simulink model "x_rx_reorder"  (R2012b)
(part 2 of 28)

      |         error('%d field names specified, but %d binary pts?', numios, length(current_bins));
      |     end
      | end
  pkt_reord_cnt1 : Subsystem  Tag=xps:sw_reg  AncestorBlock=xps_library/software register  mask(swreg){mode=one value, io_dir=To Processor, io_delay=1, sample_period=1, names=reg, bitwidths=32, arith_types=0, bin_pts=0, sim_port=off, show_format=off}
      mask prompts: io_dir "I/O direction"; io_delay "I/O delay"; sample_period "Sample period"; names "Name:"; bitwidths "Bitwidth:"; arith_types "Type (ufix=0, fix=1, bool=2):"; bin_pts "Binary pt:"; sim_port "Provide sim input/output?"; show_format "Print format string?"
      mask init:
      | swreg_init(gcb)
      settings: AttributesFormatString=1output
      mask TypeOptions mode: one value | fields of equal size | fields of arbitrary size
      mask Callback mode: swreg_cb(gcb);
      mask TypeOptions io_dir: To Processor | From Processor
      mask Callback io_dir:
      | mask_enables = get_param(gcb, 'MaskEnables');
      | mask_names = get_param(gcb, 'MaskNames');
      | if strcmp(get_param(gcb, 'io_dir'), 'To Processor'),
      |     mask_enables{ismember(mask_names, 'sample_period')} = 'off';
      | else
      |     mask_enables{ismember(mask_names, 'sample_period')} = 'on';
      | end
      | set_param(gcb, 'MaskEnables', mask_enables);
      mask Callback bitwidths:
      | blk = gcb;
      | mode = get_param(blk, 'mode');
      | current_widths = eval(get_param(blk, 'bitwidths'));
      | if (strcmp(mode, 'one value') || strcmp(mode, 'fields of equal size')) && (length(current_widths) > 1),
      |     error('Only one width may be specified for this mode.');
      | elseif strcmp(mode, 'fields of arbitrary size')
      |     current_names = textscan(strtrim(strrep(strrep(get_param(blk, 'names'), ']', ''), '[', '')), '%s');
      |     current_names = current_names{1};
      |     numios = length(current_names);
      |     if length(current_widths) ~= numios,
      |         error('%d field names specified, but %d widths?', numios, length(current_widths));
      |     end
      | end
      | total_width = 0;
      | for ctr = 1 : length(current_widths),
      |     total_width = total_width + current_widths(ctr);
      | end
      | if total_width > 32,
      |     error('Total width must be 32 or less, set to %d.', total_width);
      | end
      mask Callback arith_types:
      | blk = gcb;
      | mode = get_param(blk, 'mode');
      | current_types = eval(get_param(blk, 'arith_types'));
      | numios = length(current_types);
      | if (strcmp(mode, 'one value') || strcmp(mode, 'fields of equal size')) && (length(current_types) > 1),
      |     error('Only one type may be specified for this mode.');
      | elseif strcmp(mode, 'fields of arbitrary size')
      |     current_names = textscan(strtrim(strrep(strrep(get_param(blk, 'names'), ']', ''), '[', '')), '%s');
      |     current_names = current_names{1};
      |     numios = length(current_names);
      |     if length(current_types) ~= numios,
      |         error('%d field names specified, but %d types?', numios, length(current_types));
      |     end
      | end
      | problem = 0;
      | for ctr = 1 : numios,
      |     t = current_types(ctr);
      |     if (t < 0) || (t > 2),
      |         problem = t;
      |         ctr = numios + 1;
      |     end
      | end
      | if problem ~= 0,
      |     error('Type cannot be %i, must be 0, 1 or 2.', problem);
      | end
      mask Callback bin_pts:
      | blk = gcb;
      | mode = get_param(blk, 'mode');
      | current_bins = eval(get_param(blk, 'bin_pts'));
      | if (strcmp(mode, 'one value') || strcmp(mode, 'fields of equal size')) && (length(current_bins) > 1),
      |     error('Only one binary pt may be specified for this mode.');
      | elseif strcmp(mode, 'fields of arbitrary size')
      |     current_names = textscan(strtrim(strrep(strrep(get_param(blk, 'names'), ']', ''), '[', '')), '%s');
      |     current_names = current_names{1};
      |     numios = length(current_names);
      |     if length(current_bins) ~= numios,
      |         error('%d field names specified, but %d binary pts?', numios, length(current_bins));
      |     end
      | end
  pkt_reord_cnt2 : Subsystem  Tag=xps:sw_reg  AncestorBlock=xps_library/software register  mask(swreg){mode=one value, io_dir=To Processor, io_delay=1, sample_period=1, names=reg, bitwidths=32, arith_types=0, bin_pts=0, sim_port=off, show_format=off}
      mask prompts: io_dir "I/O direction"; io_delay "I/O delay"; sample_period "Sample period"; names "Name:"; bitwidths "Bitwidth:"; arith_types "Type (ufix=0, fix=1, bool=2):"; bin_pts "Binary pt:"; sim_port "Provide sim input/output?"; show_format "Print format string?"
      mask init:
      | swreg_init(gcb)
      settings: AttributesFormatString=1output
      mask TypeOptions mode: one value | fields of equal size | fields of arbitrary size
      mask Callback mode: swreg_cb(gcb);
      mask TypeOptions io_dir: To Processor | From Processor
      mask Callback io_dir:
      | mask_enables = get_param(gcb, 'MaskEnables');
      | mask_names = get_param(gcb, 'MaskNames');
      | if strcmp(get_param(gcb, 'io_dir'), 'To Processor'),
      |     mask_enables{ismember(mask_names, 'sample_period')} = 'off';
      | else
      |     mask_enables{ismember(mask_names, 'sample_period')} = 'on';
      | end
      | set_param(gcb, 'MaskEnables', mask_enables);
      mask Callback bitwidths:
      | blk = gcb;
      | mode = get_param(blk, 'mode');
      | current_widths = eval(get_param(blk, 'bitwidths'));
      | if (strcmp(mode, 'one value') || strcmp(mode, 'fields of equal size')) && (length(current_widths) > 1),
      |     error('Only one width may be specified for this mode.');
      | elseif strcmp(mode, 'fields of arbitrary size')
      |     current_names = textscan(strtrim(strrep(strrep(get_param(blk, 'names'), ']', ''), '[', '')), '%s');
      |     current_names = current_names{1};
      |     numios = length(current_names);
      |     if length(current_widths) ~= numios,
      |         error('%d field names specified, but %d widths?', numios, length(current_widths));
      |     end
      | end
      | total_width = 0;
      | for ctr = 1 : length(current_widths),
      |     total_width = total_width + current_widths(ctr);
      | end
      | if total_width > 32,
      |     error('Total width must be 32 or less, set to %d.', total_width);
      | end
      mask Callback arith_types:
      | blk = gcb;
      | mode = get_param(blk, 'mode');
      | current_types = eval(get_param(blk, 'arith_types'));
      | numios = length(current_types);
      | if (strcmp(mode, 'one value') || strcmp(mode, 'fields of equal size')) && (length(current_types) > 1),
      |     error('Only one type may be specified for this mode.');
      | elseif strcmp(mode, 'fields of arbitrary size')
      |     current_names = textscan(strtrim(strrep(strrep(get_param(blk, 'names'), ']', ''), '[', '')), '%s');
      |     current_names = current_names{1};
      |     numios = length(current_names);
      |     if length(current_types) ~= numios,
      |         error('%d field names specified, but %d types?', numios, length(current_types));
      |     end
      | end
      | problem = 0;
      | for ctr = 1 : numios,
      |     t = current_types(ctr);
      |     if (t < 0) || (t > 2),
      |         problem = t;
      |         ctr = numios + 1;
      |     end
      | end
      | if problem ~= 0,
      |     error('Type cannot be %i, must be 0, 1 or 2.', problem);
      | end
      mask Callback bin_pts:
      | blk = gcb;
      | mode = get_param(blk, 'mode');
      | current_bins = eval(get_param(blk, 'bin_pts'));
      | if (strcmp(mode, 'one value') || strcmp(mode, 'fields of equal size')) && (length(current_bins) > 1),
      |     error('Only one binary pt may be specified for this mode.');
      | elseif strcmp(mode, 'fields of arbitrary size')
      |     current_names = textscan(strtrim(strrep(strrep(get_param(blk, 'names'), ']', ''), '[', '')), '%s');
      |     current_names = current_names{1};
      |     numios = length(current_names);
      |     if length(current_bins) ~= numios,
      |         error('%d field names specified, but %d binary pts?', numios, length(current_bins));
      |     end
      | end
  pkt_reord_cnt3 : Subsystem  Tag=xps:sw_reg  AncestorBlock=xps_library/software register  mask(swreg){mode=one value, io_dir=To Processor, io_delay=1, sample_period=1, names=reg, bitwidths=32, arith_types=0, bin_pts=0, sim_port=off, show_format=off}
      mask prompts: io_dir "I/O direction"; io_delay "I/O delay"; sample_period "Sample period"; names "Name:"; bitwidths "Bitwidth:"; arith_types "Type (ufix=0, fix=1, bool=2):"; bin_pts "Binary pt:"; sim_port "Provide sim input/output?"; show_format "Print format string?"
      mask init:
      | swreg_init(gcb)
      settings: AttributesFormatString=1output
      mask TypeOptions mode: one value | fields of equal size | fields of arbitrary size
      mask Callback mode: swreg_cb(gcb);
      mask TypeOptions io_dir: To Processor | From Processor
      mask Callback io_dir:
      | mask_enables = get_param(gcb, 'MaskEnables');
      | mask_names = get_param(gcb, 'MaskNames');
      | if strcmp(get_param(gcb, 'io_dir'), 'To Processor'),
      |     mask_enables{ismember(mask_names, 'sample_period')} = 'off';
      | else
      |     mask_enables{ismember(mask_names, 'sample_period')} = 'on';
      | end
      | set_param(gcb, 'MaskEnables', mask_enables);
      mask Callback bitwidths:
      | blk = gcb;
      | mode = get_param(blk, 'mode');
      | current_widths = eval(get_param(blk, 'bitwidths'));
      | if (strcmp(mode, 'one value') || strcmp(mode, 'fields of equal size')) && (length(current_widths) > 1),
      |     error('Only one width may be specified for this mode.');
      | elseif strcmp(mode, 'fields of arbitrary size')
      |     current_names = textscan(strtrim(strrep(strrep(get_param(blk, 'names'), ']', ''), '[', '')), '%s');
      |     current_names = current_names{1};
      |     numios = length(current_names);
      |     if length(current_widths) ~= numios,
      |         error('%d field names specified, but %d widths?', numios, length(current_widths));
      |     end
      | end
      | total_width = 0;
      | for ctr = 1 : length(current_widths),
      |     total_width = total_width + current_widths(ctr);
      | end
      | if total_width > 32,
      |     error('Total width must be 32 or less, set to %d.', total_width);
      | end
      mask Callback arith_types:
      | blk = gcb;
      | mode = get_param(blk, 'mode');
      | current_types = eval(get_param(blk, 'arith_types'));
      | numios = length(current_types);
      | if (strcmp(mode, 'one value') || strcmp(mode, 'fields of equal size')) && (length(current_types) > 1),
      |     error('Only one type may be specified for this mode.');
      | elseif strcmp(mode, 'fields of arbitrary size')
      |     current_names = textscan(strtrim(strrep(strrep(get_param(blk, 'names'), ']', ''), '[', '')), '%s');
      |     current_names = current_names{1};
      |     numios = length(current_names);
      |     if length(current_types) ~= numios,
      |         error('%d field names specified, but %d types?', numios, length(current_types));
      |     end
      | end
      | problem = 0;
      | for ctr = 1 : numios,
      |     t = current_types(ctr);
      |     if (t < 0) || (t > 2),
      |         problem = t;
      |         ctr = numios + 1;
      |     end
      | end
      | if problem ~= 0,
      |     error('Type cannot be %i, must be 0, 1 or 2.', problem);
      | end
      mask Callback bin_pts:
      | blk = gcb;
      | mode = get_param(blk, 'mode');
      | current_bins = eval(get_param(blk, 'bin_pts'));
      | if (strcmp(mode, 'one value') || strcmp(mode, 'fields of equal size')) && (length(current_bins) > 1),
      |     error('Only one binary pt may be specified for this mode.');
      | elseif strcmp(mode, 'fields of arbitrary size')
      |     current_names = textscan(strtrim(strrep(strrep(get_param(blk, 'names'), ']', ''), '[', '')), '%s');
      |     current_names = current_names{1};
      |     numios = length(current_names);
      |     if length(current_bins) ~= numios,
      |         error('%d field names specified, but %d binary pts?', numios, length(current_bins));
      |     end
      | end
  pkt_reord_devel0 : Subsystem  mask{ant_bits=2, xeng_bits=5, chan_bits=12, x_int_bits=8, window_bits=4, min_sync_bits=11}
      mask prompts: ant_bits "Maximum Number of Antennas (2^?):"; xeng_bits "Number of Xengines in the system (2^?)"; chan_bits "Number of frequency channels in the system (2^?)"; x_int_bits "X Engine Integration Length (2^?):"; window_bits "Number of Windows to Buffer (2^?):"; min_sync_bits "Minimum sync period (2^n)"
      mask init:
      | sync_bits=max([min_sync_bits,chan_bits+x_int_bits+ant_bits-xeng_bits]);
      | %sync_bits=chan_bits+x_int_bits+ant_bits-xeng_bits;
      | buf_bits=x_int_bits+ant_bits+window_bits-1; %64b in, 32b out.
      | fmtstr = sprintf('Sync period: 2^%d\nPayload Len: %i', sync_bits, 2^(x_int_bits - 2));
      | set_param(gcb, 'AttributesFormatString', fmtstr);
      settings: AttributesFormatString=|
      | Sync period: 2^17
      | Payload Len: 64
  pkt_reord_devel1 : Subsystem  mask{ant_bits=2, xeng_bits=5, chan_bits=12, x_int_bits=8, window_bits=4, min_sync_bits=11}
      mask prompts: ant_bits "Maximum Number of Antennas (2^?):"; xeng_bits "Number of Xengines in the system (2^?)"; chan_bits "Number of frequency channels in the system (2^?)"; x_int_bits "X Engine Integration Length (2^?):"; window_bits "Number of Windows to Buffer (2^?):"; min_sync_bits "Minimum sync period (2^n)"
      mask init:
      | sync_bits=max([min_sync_bits,chan_bits+x_int_bits+ant_bits-xeng_bits]);
      | %sync_bits=chan_bits+x_int_bits+ant_bits-xeng_bits;
      | buf_bits=x_int_bits+ant_bits+window_bits-1; %64b in, 32b out.
      | fmtstr = sprintf('Sync period: 2^%d\nPayload Len: %i',sync_bits,2^(x_int_bits - 2));
      | set_param(gcb, 'AttributesFormatString', fmtstr);
      settings: AttributesFormatString=|
      | Sync period: 2^17
      | Payload Len: 64
  pkt_reord_devel2 : Subsystem  mask{ant_bits=2, xeng_bits=5, chan_bits=12, x_int_bits=8, window_bits=4, min_sync_bits=11}
      mask prompts: ant_bits "Maximum Number of Antennas (2^?):"; xeng_bits "Number of Xengines in the system (2^?)"; chan_bits "Number of frequency channels in the system (2^?)"; x_int_bits "X Engine Integration Length (2^?):"; window_bits "Number of Windows to Buffer (2^?):"; min_sync_bits "Minimum sync period (2^n)"
      mask init: same as x_rx_reorder/pkt_reord_devel1
      settings: AttributesFormatString=|
      | Sync period: 2^17
      | Payload Len: 64
  pkt_reord_devel3 : Subsystem  mask{ant_bits=2, xeng_bits=5, chan_bits=12, x_int_bits=8, window_bits=4, min_sync_bits=11}
      mask prompts: ant_bits "Maximum Number of Antennas (2^?):"; xeng_bits "Number of Xengines in the system (2^?)"; chan_bits "Number of frequency channels in the system (2^?)"; x_int_bits "X Engine Integration Length (2^?):"; window_bits "Number of Windows to Buffer (2^?):"; min_sync_bits "Minimum sync period (2^n)"
      mask init: same as x_rx_reorder/pkt_reord_devel1
      settings: AttributesFormatString=|
      | Sync period: 2^17
      | Payload Len: 64
  pkt_reord_err0 : Subsystem  Tag=xps:sw_reg  AncestorBlock=xps_library/software register  mask(swreg){mode=one value, io_dir=To Processor, io_delay=1, sample_period=1, names=reg, bitwidths=32, arith_types=0, bin_pts=0, sim_port=off, show_format=off}
      mask prompts: io_dir "I/O direction"; io_delay "I/O delay"; sample_period "Sample period"; names "Name:"; bitwidths "Bitwidth:"; arith_types "Type (ufix=0, fix=1, bool=2):"; bin_pts "Binary pt:"; sim_port "Provide sim input/output?"; show_format "Print format string?"
      mask init:
      | swreg_init(gcb)
      settings: AttributesFormatString=1output
      mask TypeOptions mode: one value | fields of equal size | fields of arbitrary size
      mask Callback mode: swreg_cb(gcb);
      mask TypeOptions io_dir: To Processor | From Processor
      mask Callback io_dir:
      | mask_enables = get_param(gcb, 'MaskEnables');
      | mask_names = get_param(gcb, 'MaskNames');
      | if strcmp(get_param(gcb, 'io_dir'), 'To Processor'),
      |     mask_enables{ismember(mask_names, 'sample_period')} = 'off';
      | else
      |     mask_enables{ismember(mask_names, 'sample_period')} = 'on';
      | end
      | set_param(gcb, 'MaskEnables', mask_enables);
      mask Callback bitwidths:
      | blk = gcb;
      | mode = get_param(blk, 'mode');
      | current_widths = eval(get_param(blk, 'bitwidths'));
      | if (strcmp(mode, 'one value') || strcmp(mode, 'fields of equal size')) && (length(current_widths) > 1),
      |     error('Only one width may be specified for this mode.');
      | elseif strcmp(mode, 'fields of arbitrary size')
      |     current_names = textscan(strtrim(strrep(strrep(get_param(blk, 'names'), ']', ''), '[', '')), '%s');
      |     current_names = current_names{1};
      |     numios = length(current_names);
      |     if length(current_widths) ~= numios,
      |         error('%d field names specified, but %d widths?', numios, length(current_widths));
      |     end
      | end
      | total_width = 0;
      | for ctr = 1 : length(current_widths),
      |     total_width = total_width + current_widths(ctr);
      | end
      | if total_width > 32,
      |     error('Total width must be 32 or less, set to %d.', total_width);
      | end
      mask Callback arith_types:
      | blk = gcb;
      | mode = get_param(blk, 'mode');
      | current_types = eval(get_param(blk, 'arith_types'));
      | numios = length(current_types);
      | if (strcmp(mode, 'one value') || strcmp(mode, 'fields of equal size')) && (length(current_types) > 1),
      |     error('Only one type may be specified for this mode.');
      | elseif strcmp(mode, 'fields of arbitrary size')
      |     current_names = textscan(strtrim(strrep(strrep(get_param(blk, 'names'), ']', ''), '[', '')), '%s');
      |     current_names = current_names{1};
      |     numios = length(current_names);
      |     if length(current_types) ~= numios,
      |         error('%d field names specified, but %d types?', numios, length(current_types));
      |     end
      | end
      | problem = 0;
      | for ctr = 1 : numios,
      |     t = current_types(ctr);
      |     if (t < 0) || (t > 2),
      |         problem = t;
      |         ctr = numios + 1;
      |     end
      | end
      | if problem ~= 0,
      |     error('Type cannot be %i, must be 0, 1 or 2.', problem);
      | end
      mask Callback bin_pts:
      | blk = gcb;
      | mode = get_param(blk, 'mode');
      | current_bins = eval(get_param(blk, 'bin_pts'));
      | if (strcmp(mode, 'one value') || strcmp(mode, 'fields of equal size')) && (length(current_bins) > 1),
      |     error('Only one binary pt may be specified for this mode.');
      | elseif strcmp(mode, 'fields of arbitrary size')
      |     current_names = textscan(strtrim(strrep(strrep(get_param(blk, 'names'), ']', ''), '[', '')), '%s');
      |     current_names = current_names{1};
      |     numios = length(current_names);
      |     if length(current_bins) ~= numios,
      |         error('%d field names specified, but %d binary pts?', numios, length(current_bins));
      |     end
      | end
  pkt_reord_err1 : Subsystem  Tag=xps:sw_reg  AncestorBlock=xps_library/software register  mask(swreg){mode=one value, io_dir=To Processor, io_delay=1, sample_period=1, names=reg, bitwidths=32, arith_types=0, bin_pts=0, sim_port=off, show_format=off}
      mask prompts: io_dir "I/O direction"; io_delay "I/O delay"; sample_period "Sample period"; names "Name:"; bitwidths "Bitwidth:"; arith_types "Type (ufix=0, fix=1, bool=2):"; bin_pts "Binary pt:"; sim_port "Provide sim input/output?"; show_format "Print format string?"
      mask init:
      | swreg_init(gcb)
      settings: AttributesFormatString=1output
      mask TypeOptions mode: one value | fields of equal size | fields of arbitrary size
      mask Callback mode: swreg_cb(gcb);
      mask TypeOptions io_dir: To Processor | From Processor
      mask Callback io_dir:
      | mask_enables = get_param(gcb, 'MaskEnables');
      | mask_names = get_param(gcb, 'MaskNames');
      | if strcmp(get_param(gcb, 'io_dir'), 'To Processor'),
      |     mask_enables{ismember(mask_names, 'sample_period')} = 'off';
      | else
      |     mask_enables{ismember(mask_names, 'sample_period')} = 'on';
      | end
      | set_param(gcb, 'MaskEnables', mask_enables);
      mask Callback bitwidths:
      | blk = gcb;
      | mode = get_param(blk, 'mode');
      | current_widths = eval(get_param(blk, 'bitwidths'));
      | if (strcmp(mode, 'one value') || strcmp(mode, 'fields of equal size')) && (length(current_widths) > 1),
      |     error('Only one width may be specified for this mode.');
      | elseif strcmp(mode, 'fields of arbitrary size')
      |     current_names = textscan(strtrim(strrep(strrep(get_param(blk, 'names'), ']', ''), '[', '')), '%s');
      |     current_names = current_names{1};
      |     numios = length(current_names);
      |     if length(current_widths) ~= numios,
      |         error('%d field names specified, but %d widths?', numios, length(current_widths));
      |     end
      | end
      | total_width = 0;
      | for ctr = 1 : length(current_widths),
      |     total_width = total_width + current_widths(ctr);
      | end
      | if total_width > 32,
      |     error('Total width must be 32 or less, set to %d.', total_width);
      | end
      mask Callback arith_types:
      | blk = gcb;
      | mode = get_param(blk, 'mode');
      | current_types = eval(get_param(blk, 'arith_types'));
      | numios = length(current_types);
      | if (strcmp(mode, 'one value') || strcmp(mode, 'fields of equal size')) && (length(current_types) > 1),
      |     error('Only one type may be specified for this mode.');
      | elseif strcmp(mode, 'fields of arbitrary size')
      |     current_names = textscan(strtrim(strrep(strrep(get_param(blk, 'names'), ']', ''), '[', '')), '%s');
      |     current_names = current_names{1};
      |     numios = length(current_names);
      |     if length(current_types) ~= numios,
      |         error('%d field names specified, but %d types?', numios, length(current_types));
      |     end
      | end
      | problem = 0;
      | for ctr = 1 : numios,
      |     t = current_types(ctr);
      |     if (t < 0) || (t > 2),
      |         problem = t;
      |         ctr = numios + 1;
      |     end
      | end
      | if problem ~= 0,
      |     error('Type cannot be %i, must be 0, 1 or 2.', problem);
      | end
      mask Callback bin_pts:
      | blk = gcb;
      | mode = get_param(blk, 'mode');
      | current_bins = eval(get_param(blk, 'bin_pts'));
      | if (strcmp(mode, 'one value') || strcmp(mode, 'fields of equal size')) && (length(current_bins) > 1),
      |     error('Only one binary pt may be specified for this mode.');
      | elseif strcmp(mode, 'fields of arbitrary size')
      |     current_names = textscan(strtrim(strrep(strrep(get_param(blk, 'names'), ']', ''), '[', '')), '%s');
      |     current_names = current_names{1};
      |     numios = length(current_names);
      |     if length(current_bins) ~= numios,
      |         error('%d field names specified, but %d binary pts?', numios, length(current_bins));
      |     end
      | end
  pkt_reord_err2 : Subsystem  Tag=xps:sw_reg  AncestorBlock=xps_library/software register  mask(swreg){mode=one value, io_dir=To Processor, io_delay=1, sample_period=1, names=reg, bitwidths=32, arith_types=0, bin_pts=0, sim_port=off, show_format=off}
      mask prompts: io_dir "I/O direction"; io_delay "I/O delay"; sample_period "Sample period"; names "Name:"; bitwidths "Bitwidth:"; arith_types "Type (ufix=0, fix=1, bool=2):"; bin_pts "Binary pt:"; sim_port "Provide sim input/output?"; show_format "Print format string?"
      mask init:
      | swreg_init(gcb)
      settings: AttributesFormatString=1output
      mask TypeOptions mode: one value | fields of equal size | fields of arbitrary size
      mask Callback mode: swreg_cb(gcb);
      mask TypeOptions io_dir: To Processor | From Processor
      mask Callback io_dir:
      | mask_enables = get_param(gcb, 'MaskEnables');
      | mask_names = get_param(gcb, 'MaskNames');
      | if strcmp(get_param(gcb, 'io_dir'), 'To Processor'),
      |     mask_enables{ismember(mask_names, 'sample_period')} = 'off';
      | else
      |     mask_enables{ismember(mask_names, 'sample_period')} = 'on';
      | end
      | set_param(gcb, 'MaskEnables', mask_enables);
      mask Callback bitwidths:
      | blk = gcb;
      | mode = get_param(blk, 'mode');
      | current_widths = eval(get_param(blk, 'bitwidths'));
      | if (strcmp(mode, 'one value') || strcmp(mode, 'fields of equal size')) && (length(current_widths) > 1),
      |     error('Only one width may be specified for this mode.');
      | elseif strcmp(mode, 'fields of arbitrary size')
      |     current_names = textscan(strtrim(strrep(strrep(get_param(blk, 'names'), ']', ''), '[', '')), '%s');
      |     current_names = current_names{1};
      |     numios = length(current_names);
      |     if length(current_widths) ~= numios,
      |         error('%d field names specified, but %d widths?', numios, length(current_widths));
      |     end
      | end
      | total_width = 0;
      | for ctr = 1 : length(current_widths),
      |     total_width = total_width + current_widths(ctr);
      | end
      | if total_width > 32,
      |     error('Total width must be 32 or less, set to %d.', total_width);
      | end
      mask Callback arith_types:
      | blk = gcb;
      | mode = get_param(blk, 'mode');
      | current_types = eval(get_param(blk, 'arith_types'));
      | numios = length(current_types);
      | if (strcmp(mode, 'one value') || strcmp(mode, 'fields of equal size')) && (length(current_types) > 1),
      |     error('Only one type may be specified for this mode.');
      | elseif strcmp(mode, 'fields of arbitrary size')
      |     current_names = textscan(strtrim(strrep(strrep(get_param(blk, 'names'), ']', ''), '[', '')), '%s');
      |     current_names = current_names{1};
      |     numios = length(current_names);
      |     if length(current_types) ~= numios,
      |         error('%d field names specified, but %d types?', numios, length(current_types));
      |     end
      | end
      | problem = 0;
      | for ctr = 1 : numios,
      |     t = current_types(ctr);
      |     if (t < 0) || (t > 2),
      |         problem = t;
      |         ctr = numios + 1;
      |     end
      | end
      | if problem ~= 0,
      |     error('Type cannot be %i, must be 0, 1 or 2.', problem);
      | end
      mask Callback bin_pts:
      | blk = gcb;
      | mode = get_param(blk, 'mode');
      | current_bins = eval(get_param(blk, 'bin_pts'));
      | if (strcmp(mode, 'one value') || strcmp(mode, 'fields of equal size')) && (length(current_bins) > 1),
      |     error('Only one binary pt may be specified for this mode.');
      | elseif strcmp(mode, 'fields of arbitrary size')
      |     current_names = textscan(strtrim(strrep(strrep(get_param(blk, 'names'), ']', ''), '[', '')), '%s');
      |     current_names = current_names{1};
      |     numios = length(current_names);
      |     if length(current_bins) ~= numios,
      |         error('%d field names specified, but %d binary pts?', numios, length(current_bins));
      |     end
      | end
  pkt_reord_err3 : Subsystem  Tag=xps:sw_reg  AncestorBlock=xps_library/software register  mask(swreg){mode=one value, io_dir=To Processor, io_delay=1, sample_period=1, names=reg, bitwidths=32, arith_types=0, bin_pts=0, sim_port=off, show_format=off}
      mask prompts: io_dir "I/O direction"; io_delay "I/O delay"; sample_period "Sample period"; names "Name:"; bitwidths "Bitwidth:"; arith_types "Type (ufix=0, fix=1, bool=2):"; bin_pts "Binary pt:"; sim_port "Provide sim input/output?"; show_format "Print format string?"
      mask init:
      | swreg_init(gcb)
      settings: AttributesFormatString=1output
      mask TypeOptions mode: one value | fields of equal size | fields of arbitrary size
      mask Callback mode: swreg_cb(gcb);
      mask TypeOptions io_dir: To Processor | From Processor
      mask Callback io_dir:
      | mask_enables = get_param(gcb, 'MaskEnables');
      | mask_names = get_param(gcb, 'MaskNames');
      | if strcmp(get_param(gcb, 'io_dir'), 'To Processor'),
      |     mask_enables{ismember(mask_names, 'sample_period')} = 'off';
      | else
      |     mask_enables{ismember(mask_names, 'sample_period')} = 'on';
      | end
      | set_param(gcb, 'MaskEnables', mask_enables);
      mask Callback bitwidths:
      | blk = gcb;
      | mode = get_param(blk, 'mode');
      | current_widths = eval(get_param(blk, 'bitwidths'));
      | if (strcmp(mode, 'one value') || strcmp(mode, 'fields of equal size')) && (length(current_widths) > 1),
      |     error('Only one width may be specified for this mode.');
      | elseif strcmp(mode, 'fields of arbitrary size')
      |     current_names = textscan(strtrim(strrep(strrep(get_param(blk, 'names'), ']', ''), '[', '')), '%s');
      |     current_names = current_names{1};
      |     numios = length(current_names);
      |     if length(current_widths) ~= numios,
      |         error('%d field names specified, but %d widths?', numios, length(current_widths));
      |     end
      | end
      | total_width = 0;
      | for ctr = 1 : length(current_widths),
      |     total_width = total_width + current_widths(ctr);
      | end
      | if total_width > 32,
      |     error('Total width must be 32 or less, set to %d.', total_width);
      | end
      mask Callback arith_types:
      | blk = gcb;
      | mode = get_param(blk, 'mode');
      | current_types = eval(get_param(blk, 'arith_types'));
      | numios = length(current_types);
      | if (strcmp(mode, 'one value') || strcmp(mode, 'fields of equal size')) && (length(current_types) > 1),
      |     error('Only one type may be specified for this mode.');
      | elseif strcmp(mode, 'fields of arbitrary size')
      |     current_names = textscan(strtrim(strrep(strrep(get_param(blk, 'names'), ']', ''), '[', '')), '%s');
      |     current_names = current_names{1};
      |     numios = length(current_names);
      |     if length(current_types) ~= numios,
      |         error('%d field names specified, but %d types?', numios, length(current_types));
      |     end
      | end
      | problem = 0;
      | for ctr = 1 : numios,
      |     t = current_types(ctr);
      |     if (t < 0) || (t > 2),
      |         problem = t;
      |         ctr = numios + 1;
      |     end
      | end
      | if problem ~= 0,
      |     error('Type cannot be %i, must be 0, 1 or 2.', problem);
      | end
      mask Callback bin_pts:
      | blk = gcb;
      | mode = get_param(blk, 'mode');
      | current_bins = eval(get_param(blk, 'bin_pts'));
      | if (strcmp(mode, 'one value') || strcmp(mode, 'fields of equal size')) && (length(current_bins) > 1),
      |     error('Only one binary pt may be specified for this mode.');
      | elseif strcmp(mode, 'fields of arbitrary size')
      |     current_names = textscan(strtrim(strrep(strrep(get_param(blk, 'names'), ']', ''), '[', '')), '%s');
      |     current_names = current_names{1};
      |     numios = length(current_names);
      |     if length(current_bins) ~= numios,
      |         error('%d field names specified, but %d binary pts?', numios, length(current_bins));
      |     end
      | end
  pre_process0 : Subsystem  mask{share_bits=1, xeng_bits=5, freq_bits=12}
      mask prompts: share_bits "Number of X-engines on this link (2^N)?"; xeng_bits "Number of X-engines in system (2^N)?"; freq_bits "Number of frequency channels in system (2^N)?"
  pre_process1 : Subsystem  mask{share_bits=1, xeng_bits=5, freq_bits=12}
      mask prompts: share_bits "Number of X-engines on this link (2^N)?"; xeng_bits "Number of X-engines in system (2^N)?"; freq_bits "Number of frequency channels in system (2^N)?"
  pre_process2 : Subsystem  mask{share_bits=1, xeng_bits=5, freq_bits=12}
      mask prompts: share_bits "Number of X-engines on this link (2^N)?"; xeng_bits "Number of X-engines in system (2^N)?"; freq_bits "Number of frequency channels in system (2^N)?"
  pre_process3 : Subsystem  mask{share_bits=1, xeng_bits=5, freq_bits=12}
      mask prompts: share_bits "Number of X-engines on this link (2^N)?"; xeng_bits "Number of X-engines in system (2^N)?"; freq_bits "Number of frequency channels in system (2^N)?"
  rx_cnt0 : Subsystem  Tag=xps:sw_reg  AncestorBlock=xps_library/software register  mask(swreg){mode=one value, io_dir=To Processor, io_delay=1, sample_period=1, names=reg, bitwidths=32, arith_types=0, bin_pts=0, sim_port=off, show_format=off}
      mask prompts: io_dir "I/O direction"; io_delay "I/O delay"; sample_period "Sample period"; names "Name:"; bitwidths "Bitwidth:"; arith_types "Type (ufix=0, fix=1, bool=2):"; bin_pts "Binary pt:"; sim_port "Provide sim input/output?"; show_format "Print format string?"
      mask init:
      | swreg_init(gcb)
      settings: AttributesFormatString=1output
      mask TypeOptions mode: one value | fields of equal size | fields of arbitrary size
      mask Callback mode: swreg_cb(gcb);
      mask TypeOptions io_dir: To Processor | From Processor
      mask Callback io_dir:
      | mask_enables = get_param(gcb, 'MaskEnables');
      | mask_names = get_param(gcb, 'MaskNames');
      | if strcmp(get_param(gcb, 'io_dir'), 'To Processor'),
      |     mask_enables{ismember(mask_names, 'sample_period')} = 'off';
      | else
      |     mask_enables{ismember(mask_names, 'sample_period')} = 'on';
      | end
      | set_param(gcb, 'MaskEnables', mask_enables);
      mask Callback bitwidths:
      | blk = gcb;
      | mode = get_param(blk, 'mode');
      | current_widths = eval(get_param(blk, 'bitwidths'));
      | if (strcmp(mode, 'one value') || strcmp(mode, 'fields of equal size')) && (length(current_widths) > 1),
      |     error('Only one width may be specified for this mode.');
      | elseif strcmp(mode, 'fields of arbitrary size')
      |     current_names = textscan(strtrim(strrep(strrep(get_param(blk, 'names'), ']', ''), '[', '')), '%s');
      |     current_names = current_names{1};
      |     numios = length(current_names);
      |     if length(current_widths) ~= numios,
      |         error('%d field names specified, but %d widths?', numios, length(current_widths));
      |     end
      | end
      | total_width = 0;
      | for ctr = 1 : length(current_widths),
      |     total_width = total_width + current_widths(ctr);
      | end
      | if total_width > 32,
      |     error('Total width must be 32 or less, set to %d.', total_width);
      | end
      mask Callback arith_types:
      | blk = gcb;
      | mode = get_param(blk, 'mode');
      | current_types = eval(get_param(blk, 'arith_types'));
      | numios = length(current_types);
      | if (strcmp(mode, 'one value') || strcmp(mode, 'fields of equal size')) && (length(current_types) > 1),
      |     error('Only one type may be specified for this mode.');
      | elseif strcmp(mode, 'fields of arbitrary size')
      |     current_names = textscan(strtrim(strrep(strrep(get_param(blk, 'names'), ']', ''), '[', '')), '%s');
      |     current_names = current_names{1};
      |     numios = length(current_names);
      |     if length(current_types) ~= numios,
      |         error('%d field names specified, but %d types?', numios, length(current_types));
      |     end
      | end
      | problem = 0;
      | for ctr = 1 : numios,
      |     t = current_types(ctr);
      |     if (t < 0) || (t > 2),
      |         problem = t;
      |         ctr = numios + 1;
      |     end
      | end
      | if problem ~= 0,
      |     error('Type cannot be %i, must be 0, 1 or 2.', problem);
      | end
      mask Callback bin_pts:
      | blk = gcb;
      | mode = get_param(blk, 'mode');
      | current_bins = eval(get_param(blk, 'bin_pts'));
      | if (strcmp(mode, 'one value') || strcmp(mode, 'fields of equal size')) && (length(current_bins) > 1),
      |     error('Only one binary pt may be specified for this mode.');
      | elseif strcmp(mode, 'fields of arbitrary size')
      |     current_names = textscan(strtrim(strrep(strrep(get_param(blk, 'names'), ']', ''), '[', '')), '%s');
      |     current_names = current_names{1};
      |     numios = length(current_names);
      |     if length(current_bins) ~= numios,
      |         error('%d field names specified, but %d binary pts?', numios, length(current_bins));
      |     end
      | end
  rx_cnt1 : Subsystem  Tag=xps:sw_reg  AncestorBlock=xps_library/software register  mask(swreg){mode=one value, io_dir=To Processor, io_delay=1, sample_period=1, names=reg, bitwidths=32, arith_types=0, bin_pts=0, sim_port=off, show_format=off}
      mask prompts: io_dir "I/O direction"; io_delay "I/O delay"; sample_period "Sample period"; names "Name:"; bitwidths "Bitwidth:"; arith_types "Type (ufix=0, fix=1, bool=2):"; bin_pts "Binary pt:"; sim_port "Provide sim input/output?"; show_format "Print format string?"
      mask init:
      | swreg_init(gcb)
      settings: AttributesFormatString=1output
      mask TypeOptions mode: one value | fields of equal size | fields of arbitrary size
      mask Callback mode: swreg_cb(gcb);
      mask TypeOptions io_dir: To Processor | From Processor
      mask Callback io_dir:
      | mask_enables = get_param(gcb, 'MaskEnables');
      | mask_names = get_param(gcb, 'MaskNames');
      | if strcmp(get_param(gcb, 'io_dir'), 'To Processor'),
      |     mask_enables{ismember(mask_names, 'sample_period')} = 'off';
      | else
      |     mask_enables{ismember(mask_names, 'sample_period')} = 'on';
      | end
      | set_param(gcb, 'MaskEnables', mask_enables);
      mask Callback bitwidths:
      | blk = gcb;
      | mode = get_param(blk, 'mode');
      | current_widths = eval(get_param(blk, 'bitwidths'));
      | if (strcmp(mode, 'one value') || strcmp(mode, 'fields of equal size')) && (length(current_widths) > 1),
      |     error('Only one width may be specified for this mode.');
      | elseif strcmp(mode, 'fields of arbitrary size')
      |     current_names = textscan(strtrim(strrep(strrep(get_param(blk, 'names'), ']', ''), '[', '')), '%s');
      |     current_names = current_names{1};
      |     numios = length(current_names);
      |     if length(current_widths) ~= numios,
      |         error('%d field names specified, but %d widths?', numios, length(current_widths));
      |     end
      | end
      | total_width = 0;
      | for ctr = 1 : length(current_widths),
      |     total_width = total_width + current_widths(ctr);
      | end
      | if total_width > 32,
      |     error('Total width must be 32 or less, set to %d.', total_width);
      | end
      mask Callback arith_types:
      | blk = gcb;
      | mode = get_param(blk, 'mode');
      | current_types = eval(get_param(blk, 'arith_types'));
      | numios = length(current_types);
      | if (strcmp(mode, 'one value') || strcmp(mode, 'fields of equal size')) && (length(current_types) > 1),
      |     error('Only one type may be specified for this mode.');
      | elseif strcmp(mode, 'fields of arbitrary size')
      |     current_names = textscan(strtrim(strrep(strrep(get_param(blk, 'names'), ']', ''), '[', '')), '%s');
      |     current_names = current_names{1};
      |     numios = length(current_names);
      |     if length(current_types) ~= numios,
      |         error('%d field names specified, but %d types?', numios, length(current_types));
      |     end
      | end
      | problem = 0;
      | for ctr = 1 : numios,
      |     t = current_types(ctr);
      |     if (t < 0) || (t > 2),
      |         problem = t;
      |         ctr = numios + 1;
      |     end
      | end
      | if problem ~= 0,
      |     error('Type cannot be %i, must be 0, 1 or 2.', problem);
      | end
      mask Callback bin_pts:
      | blk = gcb;
      | mode = get_param(blk, 'mode');
      | current_bins = eval(get_param(blk, 'bin_pts'));
      | if (strcmp(mode, 'one value') || strcmp(mode, 'fields of equal size')) && (length(current_bins) > 1),
      |     error('Only one binary pt may be specified for this mode.');
      | elseif strcmp(mode, 'fields of arbitrary size')
      |     current_names = textscan(strtrim(strrep(strrep(get_param(blk, 'names'), ']', ''), '[', '')), '%s');
      |     current_names = current_names{1};
      |     numios = length(current_names);
      |     if length(current_bins) ~= numios,
      |         error('%d field names specified, but %d binary pts?', numios, length(current_bins));
      |     end
      | end
  rx_err_cnt0 : Subsystem  Tag=xps:sw_reg  AncestorBlock=xps_library/software register  mask(swreg){mode=one value, io_dir=To Processor, io_delay=1, sample_period=1, names=reg, bitwidths=32, arith_types=0, bin_pts=0, sim_port=off, show_format=off}
      mask prompts: io_dir "I/O direction"; io_delay "I/O delay"; sample_period "Sample period"; names "Name:"; bitwidths "Bitwidth:"; arith_types "Type (ufix=0, fix=1, bool=2):"; bin_pts "Binary pt:"; sim_port "Provide sim input/output?"; show_format "Print format string?"
      mask init:
      | swreg_init(gcb)
      settings: AttributesFormatString=1output
      mask TypeOptions mode: one value | fields of equal size | fields of arbitrary size
      mask Callback mode: swreg_cb(gcb);
      mask TypeOptions io_dir: To Processor | From Processor
      mask Callback io_dir:
      | mask_enables = get_param(gcb, 'MaskEnables');
      | mask_names = get_param(gcb, 'MaskNames');
      | if strcmp(get_param(gcb, 'io_dir'), 'To Processor'),
      |     mask_enables{ismember(mask_names, 'sample_period')} = 'off';
      | else
      |     mask_enables{ismember(mask_names, 'sample_period')} = 'on';
      | end
      | set_param(gcb, 'MaskEnables', mask_enables);
      mask Callback bitwidths:
      | blk = gcb;
      | mode = get_param(blk, 'mode');
      | current_widths = eval(get_param(blk, 'bitwidths'));
      | if (strcmp(mode, 'one value') || strcmp(mode, 'fields of equal size')) && (length(current_widths) > 1),
      |     error('Only one width may be specified for this mode.');
      | elseif strcmp(mode, 'fields of arbitrary size')
      |     current_names = textscan(strtrim(strrep(strrep(get_param(blk, 'names'), ']', ''), '[', '')), '%s');
      |     current_names = current_names{1};
      |     numios = length(current_names);
      |     if length(current_widths) ~= numios,
      |         error('%d field names specified, but %d widths?', numios, length(current_widths));
      |     end
      | end
      | total_width = 0;
      | for ctr = 1 : length(current_widths),
      |     total_width = total_width + current_widths(ctr);
      | end
      | if total_width > 32,
      |     error('Total width must be 32 or less, set to %d.', total_width);
      | end
      mask Callback arith_types:
      | blk = gcb;
      | mode = get_param(blk, 'mode');
      | current_types = eval(get_param(blk, 'arith_types'));
      | numios = length(current_types);
      | if (strcmp(mode, 'one value') || strcmp(mode, 'fields of equal size')) && (length(current_types) > 1),
      |     error('Only one type may be specified for this mode.');
      | elseif strcmp(mode, 'fields of arbitrary size')
      |     current_names = textscan(strtrim(strrep(strrep(get_param(blk, 'names'), ']', ''), '[', '')), '%s');
      |     current_names = current_names{1};
      |     numios = length(current_names);
      |     if length(current_types) ~= numios,
      |         error('%d field names specified, but %d types?', numios, length(current_types));
      |     end
      | end
      | problem = 0;
      | for ctr = 1 : numios,
      |     t = current_types(ctr);
      |     if (t < 0) || (t > 2),
      |         problem = t;
      |         ctr = numios + 1;
      |     end
      | end
      | if problem ~= 0,
      |     error('Type cannot be %i, must be 0, 1 or 2.', problem);
      | end
      mask Callback bin_pts:
      | blk = gcb;
      | mode = get_param(blk, 'mode');
      | current_bins = eval(get_param(blk, 'bin_pts'));
      | if (strcmp(mode, 'one value') || strcmp(mode, 'fields of equal size')) && (length(current_bins) > 1),
      |     error('Only one binary pt may be specified for this mode.');
      | elseif strcmp(mode, 'fields of arbitrary size')
      |     current_names = textscan(strtrim(strrep(strrep(get_param(blk, 'names'), ']', ''), '[', '')), '%s');
      |     current_names = current_names{1};
      |     numios = length(current_names);
      |     if length(current_bins) ~= numios,
      |         error('%d field names specified, but %d binary pts?', numios, length(current_bins));
      |     end
      | end
  rx_err_cnt1 : Subsystem  Tag=xps:sw_reg  AncestorBlock=xps_library/software register  mask(swreg){mode=one value, io_dir=To Processor, io_delay=1, sample_period=1, names=reg, bitwidths=32, arith_types=0, bin_pts=0, sim_port=off, show_format=off}
      mask prompts: io_dir "I/O direction"; io_delay "I/O delay"; sample_period "Sample period"; names "Name:"; bitwidths "Bitwidth:"; arith_types "Type (ufix=0, fix=1, bool=2):"; bin_pts "Binary pt:"; sim_port "Provide sim input/output?"; show_format "Print format string?"
      mask init:
      | swreg_init(gcb)
      settings: AttributesFormatString=1output
      mask TypeOptions mode: one value | fields of equal size | fields of arbitrary size
      mask Callback mode: swreg_cb(gcb);
      mask TypeOptions io_dir: To Processor | From Processor
      mask Callback io_dir:
      | mask_enables = get_param(gcb, 'MaskEnables');
      | mask_names = get_param(gcb, 'MaskNames');
      | if strcmp(get_param(gcb, 'io_dir'), 'To Processor'),
      |     mask_enables{ismember(mask_names, 'sample_period')} = 'off';
      | else
      |     mask_enables{ismember(mask_names, 'sample_period')} = 'on';
      | end
      | set_param(gcb, 'MaskEnables', mask_enables);
      mask Callback bitwidths:
      | blk = gcb;
      | mode = get_param(blk, 'mode');
      | current_widths = eval(get_param(blk, 'bitwidths'));
      | if (strcmp(mode, 'one value') || strcmp(mode, 'fields of equal size')) && (length(current_widths) > 1),
      |     error('Only one width may be specified for this mode.');
      | elseif strcmp(mode, 'fields of arbitrary size')
      |     current_names = textscan(strtrim(strrep(strrep(get_param(blk, 'names'), ']', ''), '[', '')), '%s');
      |     current_names = current_names{1};
      |     numios = length(current_names);
      |     if length(current_widths) ~= numios,
      |         error('%d field names specified, but %d widths?', numios, length(current_widths));
      |     end
      | end
      | total_width = 0;
      | for ctr = 1 : length(current_widths),
      |     total_width = total_width + current_widths(ctr);
      | end
      | if total_width > 32,
      |     error('Total width must be 32 or less, set to %d.', total_width);
      | end
      mask Callback arith_types:
      | blk = gcb;
      | mode = get_param(blk, 'mode');
      | current_types = eval(get_param(blk, 'arith_types'));
      | numios = length(current_types);
      | if (strcmp(mode, 'one value') || strcmp(mode, 'fields of equal size')) && (length(current_types) > 1),
      |     error('Only one type may be specified for this mode.');
      | elseif strcmp(mode, 'fields of arbitrary size')
      |     current_names = textscan(strtrim(strrep(strrep(get_param(blk, 'names'), ']', ''), '[', '')), '%s');
      |     current_names = current_names{1};
      |     numios = length(current_names);
      |     if length(current_types) ~= numios,
      |         error('%d field names specified, but %d types?', numios, length(current_types));
      |     end
      | end
      | problem = 0;
      | for ctr = 1 : numios,
      |     t = current_types(ctr);
      |     if (t < 0) || (t > 2),
      |         problem = t;
      |         ctr = numios + 1;
      |     end
      | end
      | if problem ~= 0,
      |     error('Type cannot be %i, must be 0, 1 or 2.', problem);
      | end
      mask Callback bin_pts:
      | blk = gcb;
      | mode = get_param(blk, 'mode');
      | current_bins = eval(get_param(blk, 'bin_pts'));
      | if (strcmp(mode, 'one value') || strcmp(mode, 'fields of equal size')) && (length(current_bins) > 1),
      |     error('Only one binary pt may be specified for this mode.');
      | elseif strcmp(mode, 'fields of arbitrary size')
      |     current_names = textscan(strtrim(strrep(strrep(get_param(blk, 'names'), ']', ''), '[', '')), '%s');
      |     current_names = current_names{1};
      |     numios = length(current_names);
      |     if length(current_bins) ~= numios,
      |         error('%d field names specified, but %d binary pts?', numios, length(current_bins));
      |     end
      | end
  snap_reord0 : Subsystem  Tag=casper:bitsnap  AncestorBlock=casper_library_scopes/bitfield snapshot  mask(bitsnap){io_names=[sync, data, valid, time, freq, xeng_err, feng_err, adc_over, nd_on], io_widths=[1,32,1,48,42,1,1,1,1], io_bps=[0,0,0,0,0,0,0,0,0], io_types=[2,0,2,0,0,2,2,2,2], snap_storage=bram, snap_dram_dimm=2, snap_dram_clock=250, snap_nsamples=10, snap_data_width=128, snap_offset=on, snap_circap=on, snap_value=off, snap_use_dsp48=on, snap_delay=0, extra_names=[c d], extra_widths=[30 2], extra_bps=[0 0], extra_types=[0 0]}
      mask prompts: io_names "Names [msb...lsb]"; io_widths "Widths [msb...lsb]"; io_bps "Binary pts [msb...lsb]"; io_types "Data types [msb...lsb], ufix=0, fix=1, bool=2"; snap_storage "Storage medium"; snap_dram_dimm "DRAM dimm"; snap_dram_clock "DRAM clock rate"; snap_nsamples "Number of Samples (2^?)"; snap_data_width "Data width"; snap_offset "Start delay support"; snap_circap "Circular capture support"; snap_value "Extra value capture support"; snap_use_dsp48 "Use DSP48s to implement counters"; snap_delay "Pre-snapshot delay"; extra_names "Names [msb...lsb]"; extra_widths "Widths [msb...lsb]"; extra_bps "Binary pts [msb...lsb]"; extra_types "Data types [msb...lsb], ufix=0, fix=1, bool=2"
      mask help:
      | A wrapped snapshot block. Allows specification of inputs to a snapblock word so the toolflow can automatically set up the scope.
      | See documentation for snapshot for explanation of parameters.
      mask init:
      | bitsnap_init(gcb);
      mask TypeOptions snap_storage: bram | dram
      mask Callback snap_storage: bitsnap_callback();
      mask TypeOptions snap_dram_dimm: 1 | 2 | 3 | 4
      mask TypeOptions snap_dram_clock: 200 | 250 | 266 | 300 | 333
      mask TypeOptions snap_data_width: 8 | 16 | 32 | 64 | 128
      mask Callback snap_value: bitsnap_callback();
  snap_unpack0 : Subsystem  Tag=casper:bitsnap  AncestorBlock=casper_library_scopes/bitfield snapshot  mask(bitsnap){io_names=[data valid eof time feng_id freq adc_over spead_err dest_err fft_err feng_rx_err nd_en chksum_err feng_qdr_err], io_widths=[64,1,1,31,7,16,1,1,1,1,1,1,1,1], io_bps=[0,0,0,0,0,0,0,0,0,0,0,0,0,0], io_types=[0,2,2,0,0,0,2,2,2,2,2,2,2,2], snap_storage=bram, snap_dram_dimm=2, snap_dram_clock=250, snap_nsamples=12, snap_data_width=128, snap_offset=on, snap_circap=on, snap_value=off, snap_use_dsp48=on, snap_delay=0, extra_names=[c d], extra_widths=[30 2], extra_bps=[0 0], extra_types=[0 0]}
      mask prompts: io_names "Names [msb...lsb]"; io_widths "Widths [msb...lsb]"; io_bps "Binary pts [msb...lsb]"; io_types "Data types [msb...lsb], ufix=0, fix=1, bool=2"; snap_storage "Storage medium"; snap_dram_dimm "DRAM dimm"; snap_dram_clock "DRAM clock rate"; snap_nsamples "Number of Samples (2^?)"; snap_data_width "Data width"; snap_offset "Start delay support"; snap_circap "Circular capture support"; snap_value "Extra value capture support"; snap_use_dsp48 "Use DSP48s to implement counters"; snap_delay "Pre-snapshot delay"; extra_names "Names [msb...lsb]"; extra_widths "Widths [msb...lsb]"; extra_bps "Binary pts [msb...lsb]"; extra_types "Data types [msb...lsb], ufix=0, fix=1, bool=2"
      mask help:
      | A wrapped snapshot block. Allows specification of inputs to a snapblock word so the toolflow can automatically set up the scope.
      | See documentation for snapshot for explanation of parameters.
      mask init:
      | bitsnap_init(gcb);
      mask TypeOptions snap_storage: bram | dram
      mask Callback snap_storage: bitsnap_callback();
      mask TypeOptions snap_dram_dimm: 1 | 2 | 3 | 4
      mask TypeOptions snap_dram_clock: 200 | 250 | 266 | 300 | 333
      mask TypeOptions snap_data_width: 8 | 16 | 32 | 64 | 128
      mask Callback snap_value: bitsnap_callback();
  snap_unpack1 : Subsystem  Tag=casper:bitsnap  AncestorBlock=casper_library_scopes/bitfield snapshot  mask(bitsnap){io_names=[data valid eof time feng_id freq adc_over spead_err dest_err fft_err feng_rx_err nd_en chksum_err feng_qdr_err], io_widths=[64,1,1,31,7,16,1,1,1,1,1,1,1,1], io_bps=[0,0,0,0,0,0,0,0,0,0,0,0,0,0], io_types=[0,2,2,0,0,0,2,2,2,2,2,2,2,2], snap_storage=bram, snap_dram_dimm=2, snap_dram_clock=250, snap_nsamples=12, snap_data_width=128, snap_offset=on, snap_circap=on, snap_value=off, snap_use_dsp48=on, snap_delay=0, extra_names=[c d], extra_widths=[30 2], extra_bps=[0 0], extra_types=[0 0]}
      mask prompts: io_names "Names [msb...lsb]"; io_widths "Widths [msb...lsb]"; io_bps "Binary pts [msb...lsb]"; io_types "Data types [msb...lsb], ufix=0, fix=1, bool=2"; snap_storage "Storage medium"; snap_dram_dimm "DRAM dimm"; snap_dram_clock "DRAM clock rate"; snap_nsamples "Number of Samples (2^?)"; snap_data_width "Data width"; snap_offset "Start delay support"; snap_circap "Circular capture support"; snap_value "Extra value capture support"; snap_use_dsp48 "Use DSP48s to implement counters"; snap_delay "Pre-snapshot delay"; extra_names "Names [msb...lsb]"; extra_widths "Widths [msb...lsb]"; extra_bps "Binary pts [msb...lsb]"; extra_types "Data types [msb...lsb], ufix=0, fix=1, bool=2"
      mask help:
      | A wrapped snapshot block. Allows specification of inputs to a snapblock word so the toolflow can automatically set up the scope.
      | See documentation for snapshot for explanation of parameters.
      mask init:
      | bitsnap_init(gcb);
      mask TypeOptions snap_storage: bram | dram
      mask Callback snap_storage: bitsnap_callback();
      mask TypeOptions snap_dram_dimm: 1 | 2 | 3 | 4
      mask TypeOptions snap_dram_clock: 200 | 250 | 266 | 300 | 333
      mask TypeOptions snap_data_width: 8 | 16 | 32 | 64 | 128
      mask Callback snap_value: bitsnap_callback();
  snap_unpack2 : Subsystem  Tag=casper:bitsnap  AncestorBlock=casper_library_scopes/bitfield snapshot  mask(bitsnap){io_names=[data valid eof time feng_id freq adc_over spead_err dest_err fft_err feng_rx_err nd_en chksum_err feng_qdr_err], io_widths=[64,1,1,31,7,16,1,1,1,1,1,1,1,1], io_bps=[0,0,0,0,0,0,0,0,0,0,0,0,0,0], io_types=[0,2,2,0,0,0,2,2,2,2,2,2,2,2], snap_storage=bram, snap_dram_dimm=2, snap_dram_clock=250, snap_nsamples=12, snap_data_width=128, snap_offset=on, snap_circap=on, snap_value=off, snap_use_dsp48=on, snap_delay=0, extra_names=[c d], extra_widths=[30 2], extra_bps=[0 0], extra_types=[0 0]}
      mask prompts: io_names "Names [msb...lsb]"; io_widths "Widths [msb...lsb]"; io_bps "Binary pts [msb...lsb]"; io_types "Data types [msb...lsb], ufix=0, fix=1, bool=2"; snap_storage "Storage medium"; snap_dram_dimm "DRAM dimm"; snap_dram_clock "DRAM clock rate"; snap_nsamples "Number of Samples (2^?)"; snap_data_width "Data width"; snap_offset "Start delay support"; snap_circap "Circular capture support"; snap_value "Extra value capture support"; snap_use_dsp48 "Use DSP48s to implement counters"; snap_delay "Pre-snapshot delay"; extra_names "Names [msb...lsb]"; extra_widths "Widths [msb...lsb]"; extra_bps "Binary pts [msb...lsb]"; extra_types "Data types [msb...lsb], ufix=0, fix=1, bool=2"
      mask help:
      | A wrapped snapshot block. Allows specification of inputs to a snapblock word so the toolflow can automatically set up the scope.
      | See documentation for snapshot for explanation of parameters.
      mask init:
      | bitsnap_init(gcb);
      mask TypeOptions snap_storage: bram | dram
      mask Callback snap_storage: bitsnap_callback();
      mask TypeOptions snap_dram_dimm: 1 | 2 | 3 | 4
      mask TypeOptions snap_dram_clock: 200 | 250 | 266 | 300 | 333
      mask TypeOptions snap_data_width: 8 | 16 | 32 | 64 | 128
      mask Callback snap_value: bitsnap_callback();
  snap_unpack3 : Subsystem  Tag=casper:bitsnap  AncestorBlock=casper_library_scopes/bitfield snapshot  mask(bitsnap){io_names=[data valid eof time feng_id freq adc_over spead_err dest_err fft_err feng_rx_err nd_en chksum_err feng_qdr_err], io_widths=[64,1,1,31,7,16,1,1,1,1,1,1,1,1], io_bps=[0,0,0,0,0,0,0,0,0,0,0,0,0,0], io_types=[0,2,2,0,0,0,2,2,2,2,2,2,2,2], snap_storage=bram, snap_dram_dimm=2, snap_dram_clock=250, snap_nsamples=12, snap_data_width=128, snap_offset=on, snap_circap=on, snap_value=off, snap_use_dsp48=on, snap_delay=0, extra_names=[c d], extra_widths=[30 2], extra_bps=[0 0], extra_types=[0 0]}
      mask prompts: io_names "Names [msb...lsb]"; io_widths "Widths [msb...lsb]"; io_bps "Binary pts [msb...lsb]"; io_types "Data types [msb...lsb], ufix=0, fix=1, bool=2"; snap_storage "Storage medium"; snap_dram_dimm "DRAM dimm"; snap_dram_clock "DRAM clock rate"; snap_nsamples "Number of Samples (2^?)"; snap_data_width "Data width"; snap_offset "Start delay support"; snap_circap "Circular capture support"; snap_value "Extra value capture support"; snap_use_dsp48 "Use DSP48s to implement counters"; snap_delay "Pre-snapshot delay"; extra_names "Names [msb...lsb]"; extra_widths "Widths [msb...lsb]"; extra_bps "Binary pts [msb...lsb]"; extra_types "Data types [msb...lsb], ufix=0, fix=1, bool=2"
      mask help:
      | A wrapped snapshot block. Allows specification of inputs to a snapblock word so the toolflow can automatically set up the scope.
      | See documentation for snapshot for explanation of parameters.
      mask init:
      | bitsnap_init(gcb);
      mask TypeOptions snap_storage: bram | dram
      mask Callback snap_storage: bitsnap_callback();
      mask TypeOptions snap_dram_dimm: 1 | 2 | 3 | 4
      mask TypeOptions snap_dram_clock: 200 | 250 | 266 | 300 | 333
      mask TypeOptions snap_data_width: 8 | 16 | 32 | 64 | 128
      mask Callback snap_value: bitsnap_callback();
  spead_unpack0 : Subsystem  Tag=casper:spead_unpack  AncestorBlock=casper_library_communications/spead_unpack  mask(spead_unpack_mask){payload_length=128, header_ids=[hex2dec('1600'),hex2dec('4101'),hex2dec('4102'), hex2dec('4103')], spead_msw=64, spead_lsw=48, spead_version=4, combine_errors=on}
      mask prompts: payload_length "Payload length in 64-bit words"; header_ids "SPEAD header IDs (decimal)"; spead_msw "SPEAD Flavour (MSw)"; spead_lsw "SPEAD Flavour (LSw)"; spead_version "SPEAD version"; combine_errors "Combine error flags"
      mask help: This block receives a 64-bit-word stream that contains a SPEAD stream. It checks the SPEAD headers are being correctly received. It presents the user with all headers on the first valid cycle of data along with a flag to indicate a header or packet-length error.
      mask init:
      | spead_unpack_init(gcb)
  spead_unpack1 : Subsystem  Tag=casper:spead_unpack  AncestorBlock=casper_library_communications/spead_unpack  mask(spead_unpack_mask){payload_length=128, header_ids=[hex2dec('1600'),hex2dec('4101'),hex2dec('4102'), hex2dec('4103')], spead_msw=64, spead_lsw=48, spead_version=4, combine_errors=on}
      mask prompts: payload_length "Payload length in 64-bit words"; header_ids "SPEAD header IDs (decimal)"; spead_msw "SPEAD Flavour (MSw)"; spead_lsw "SPEAD Flavour (LSw)"; spead_version "SPEAD version"; combine_errors "Combine error flags"
      mask help: This block receives a 64-bit-word stream that contains a SPEAD stream. It checks the SPEAD headers are being correctly received. It presents the user with all headers on the first valid cycle of data along with a flag to indicate a header or packet-length error.
      mask init:
      | spead_unpack_init(gcb)
  tvg_select : Subsystem  Tag=xps:sw_reg  AncestorBlock=xps_library/software register  mask(swreg){mode=fields of arbitrary size, io_dir=From Processor, io_delay=1, sample_period=1, names=[xaui descramble xeng vacc], bitwidths=[1 2 2 6], arith_types=[0 0 0 0], bin_pts=[0 0 0 0], sim_port=off, show_format=off}
      mask prompts: io_dir "I/O direction"; io_delay "I/O delay"; sample_period "Sample period"; names "Names [msb ... lsb]:"; bitwidths "Bitwidths [msb ... lsb]:"; arith_types "Types (ufix=0, fix=1, bool=2) [msb ... lsb]:"; bin_pts "Binary pts [msb ... lsb]:"; sim_port "Provide sim input/output?"; show_format "Print format string?"
      mask init:
      | swreg_init(gcb)
      settings: AttributesFormatString=4 inputs
      mask TypeOptions mode: one value | fields of equal size | fields of arbitrary size
      mask Callback mode: swreg_cb(gcb);
      mask TypeOptions io_dir: To Processor | From Processor
      mask Callback io_dir:
      | mask_enables = get_param(gcb, 'MaskEnables');
      | mask_names = get_param(gcb, 'MaskNames');
      | if strcmp(get_param(gcb, 'io_dir'), 'To Processor'),
      |     mask_enables{ismember(mask_names, 'sample_period')} = 'off';
      | else
      |     mask_enables{ismember(mask_names, 'sample_period')} = 'on';
      | end
      | set_param(gcb, 'MaskEnables', mask_enables);
      mask Callback bitwidths:
      | blk = gcb;
      | mode = get_param(blk, 'mode');
      | current_widths = eval(get_param(blk, 'bitwidths'));
      | if (strcmp(mode, 'one value') || strcmp(mode, 'fields of equal size')) && (length(current_widths) > 1),
      |     error('Only one width may be specified for this mode.');
      | elseif strcmp(mode, 'fields of arbitrary size')
      |     current_names = textscan(strtrim(strrep(strrep(get_param(blk, 'names'), ']', ''), '[', '')), '%s');
      |     current_names = current_names{1};
      |     numios = length(current_names);
      |     if length(current_widths) ~= numios,
      |         error('%d field names specified, but %d widths?', numios, length(current_widths));
      |     end
      | end
      | total_width = 0;
      | for ctr = 1 : length(current_widths),
      |     total_width = total_width + current_widths(ctr);
      | end
      | if total_width > 32,
      |     error('Total width must be 32 or less, set to %d.', total_width);
      | end
      mask Callback arith_types:
      | blk = gcb;
      | mode = get_param(blk, 'mode');
      | current_types = eval(get_param(blk, 'arith_types'));
      | numios = length(current_types);
      | if (strcmp(mode, 'one value') || strcmp(mode, 'fields of equal size')) && (length(current_types) > 1),
      |     error('Only one type may be specified for this mode.');
      | elseif strcmp(mode, 'fields of arbitrary size')
      |     current_names = textscan(strtrim(strrep(strrep(get_param(blk, 'names'), ']', ''), '[', '')), '%s');
      |     current_names = current_names{1};
      |     numios = length(current_names);
      |     if length(current_types) ~= numios,
      |         error('%d field names specified, but %d types?', numios, length(current_types));
      |     end
      | end
      | problem = 0;
      | for ctr = 1 : numios,
      |     t = current_types(ctr);
      |     if (t < 0) || (t > 2),
      |         problem = t;
      |         ctr = numios + 1;
      |     end
      | end
      | if problem ~= 0,
      |     error('Type cannot be %i, must be 0, 1 or 2.', problem);
      | end
      mask Callback bin_pts:
      | blk = gcb;
      | mode = get_param(blk, 'mode');
      | current_bins = eval(get_param(blk, 'bin_pts'));
      | if (strcmp(mode, 'one value') || strcmp(mode, 'fields of equal size')) && (length(current_bins) > 1),
      |     error('Only one binary pt may be specified for this mode.');
      | elseif strcmp(mode, 'fields of arbitrary size')
      |     current_names = textscan(strtrim(strrep(strrep(get_param(blk, 'names'), ']', ''), '[', '')), '%s');
      |     current_names = current_names{1};
      |     numios = length(current_names);
      |     if length(current_bins) ~= numios,
      |         error('%d field names specified, but %d binary pts?', numios, length(current_bins));
      |     end
      | end
  vacc_time_lsw : Subsystem  Tag=xps:sw_reg  AncestorBlock=xps_library/software register  mask(swreg){mode=one value, io_dir=From Processor, io_delay=1, sample_period=1, names=reg, bitwidths=32, arith_types=0, bin_pts=0, sim_port=on, show_format=off}
      mask prompts: io_dir "I/O direction"; io_delay "I/O delay"; sample_period "Sample period"; names "Name:"; bitwidths "Bitwidth:"; arith_types "Type (ufix=0, fix=1, bool=2):"; bin_pts "Binary pt:"; sim_port "Provide sim input/output?"; show_format "Print format string?"
      mask init:
      | swreg_init(gcb)
      settings: AttributesFormatString=1input
      mask TypeOptions mode: one value | fields of equal size | fields of arbitrary size
      mask Callback mode: swreg_cb(gcb);
      mask TypeOptions io_dir: To Processor | From Processor
      mask Callback io_dir:
      | mask_enables = get_param(gcb, 'MaskEnables');
      | mask_names = get_param(gcb, 'MaskNames');
      | if strcmp(get_param(gcb, 'io_dir'), 'To Processor'),
      |     mask_enables{ismember(mask_names, 'sample_period')} = 'off';
      | else
      |     mask_enables{ismember(mask_names, 'sample_period')} = 'on';
      | end
      | set_param(gcb, 'MaskEnables', mask_enables);
      mask Callback bitwidths:
      | blk = gcb;
      | mode = get_param(blk, 'mode');
      | current_widths = eval(get_param(blk, 'bitwidths'));
      | if (strcmp(mode, 'one value') || strcmp(mode, 'fields of equal size')) && (length(current_widths) > 1),
      |     error('Only one width may be specified for this mode.');
      | elseif strcmp(mode, 'fields of arbitrary size')
      |     current_names = textscan(strtrim(strrep(strrep(get_param(blk, 'names'), ']', ''), '[', '')), '%s');
      |     current_names = current_names{1};
      |     numios = length(current_names);
      |     if length(current_widths) ~= numios,
      |         error('%d field names specified, but %d widths?', numios, length(current_widths));
      |     end
      | end
      | total_width = 0;
      | for ctr = 1 : length(current_widths),
      |     total_width = total_width + current_widths(ctr);
      | end
      | if total_width > 32,
      |     error('Total width must be 32 or less, set to %d.', total_width);
      | end
      mask Callback arith_types:
      | blk = gcb;
      | mode = get_param(blk, 'mode');
      | current_types = eval(get_param(blk, 'arith_types'));
      | numios = length(current_types);
      | if (strcmp(mode, 'one value') || strcmp(mode, 'fields of equal size')) && (length(current_types) > 1),
      |     error('Only one type may be specified for this mode.');
      | elseif strcmp(mode, 'fields of arbitrary size')
      |     current_names = textscan(strtrim(strrep(strrep(get_param(blk, 'names'), ']', ''), '[', '')), '%s');
      |     current_names = current_names{1};
      |     numios = length(current_names);
      |     if length(current_types) ~= numios,
      |         error('%d field names specified, but %d types?', numios, length(current_types));
      |     end
      | end
      | problem = 0;
      | for ctr = 1 : numios,
      |     t = current_types(ctr);
      |     if (t < 0) || (t > 2),
      |         problem = t;
      |         ctr = numios + 1;
      |     end
      | end
      | if problem ~= 0,
      |     error('Type cannot be %i, must be 0, 1 or 2.', problem);
      | end
      mask Callback bin_pts:
      | blk = gcb;
      | mode = get_param(blk, 'mode');
      | current_bins = eval(get_param(blk, 'bin_pts'));
      | if (strcmp(mode, 'one value') || strcmp(mode, 'fields of equal size')) && (length(current_bins) > 1),
      |     error('Only one binary pt may be specified for this mode.');
      | elseif strcmp(mode, 'fields of arbitrary size')
      |     current_names = textscan(strtrim(strrep(strrep(get_param(blk, 'names'), ']', ''), '[', '')), '%s');
      |     current_names = current_names{1};
      |     numios = length(current_names);
      |     if length(current_bins) ~= numios,
      |         error('%d field names specified, but %d binary pts?', numios, length(current_bins));
      |     end
      | end
  vacc_time_msw : Subsystem  Tag=xps:sw_reg  AncestorBlock=xps_library/software register  mask(swreg){mode=fields of arbitrary size, io_dir=From Processor, io_delay=1, sample_period=1, names=[arm msw], bitwidths=[1 16], arith_types=[2 0], bin_pts=[0 0], sim_port=off, show_format=on}
      mask prompts: io_dir "I/O direction"; io_delay "I/O delay"; sample_period "Sample period"; names "Names [msb ... lsb]:"; bitwidths "Bitwidths [msb ... lsb]:"; arith_types "Types (ufix=0, fix=1, bool=2) [msb ... lsb]:"; bin_pts "Binary pts [msb ... lsb]:"; sim_port "Provide sim input/output?"; show_format "Print format string?"
      mask init:
      | swreg_init(gcb)
      settings: AttributesFormatString=2 inputs:b,uf16.0,
      mask TypeOptions mode: one value | fields of equal size | fields of arbitrary size
      mask Callback mode: swreg_cb(gcb);
      mask TypeOptions io_dir: To Processor | From Processor
      mask Callback io_dir:
      | mask_enables = get_param(gcb, 'MaskEnables');
      | mask_names = get_param(gcb, 'MaskNames');
      | if strcmp(get_param(gcb, 'io_dir'), 'To Processor'),
      |     mask_enables{ismember(mask_names, 'sample_period')} = 'off';
      | else
      |     mask_enables{ismember(mask_names, 'sample_period')} = 'on';
      | end
      | set_param(gcb, 'MaskEnables', mask_enables);
      mask Callback bitwidths:
      | blk = gcb;
      | mode = get_param(blk, 'mode');
      | current_widths = eval(get_param(blk, 'bitwidths'));
      | if (strcmp(mode, 'one value') || strcmp(mode, 'fields of equal size')) && (length(current_widths) > 1),
      |     error('Only one width may be specified for this mode.');
      | elseif strcmp(mode, 'fields of arbitrary size')
      |     current_names = textscan(strtrim(strrep(strrep(get_param(blk, 'names'), ']', ''), '[', '')), '%s');
      |     current_names = current_names{1};
      |     numios = length(current_names);
      |     if length(current_widths) ~= numios,
      |         error('%d field names specified, but %d widths?', numios, length(current_widths));
      |     end
      | end
      | total_width = 0;
      | for ctr = 1 : length(current_widths),
      |     total_width = total_width + current_widths(ctr);
      | end
      | if total_width > 32,
      |     error('Total width must be 32 or less, set to %d.', total_width);
      | end
      mask Callback arith_types:
      | blk = gcb;
      | mode = get_param(blk, 'mode');
      | current_types = eval(get_param(blk, 'arith_types'));
      | numios = length(current_types);
      | if (strcmp(mode, 'one value') || strcmp(mode, 'fields of equal size')) && (length(current_types) > 1),
      |     error('Only one type may be specified for this mode.');
      | elseif strcmp(mode, 'fields of arbitrary size')
      |     current_names = textscan(strtrim(strrep(strrep(get_param(blk, 'names'), ']', ''), '[', '')), '%s');
      |     current_names = current_names{1};
      |     numios = length(current_names);
      |     if length(current_types) ~= numios,
      |         error('%d field names specified, but %d types?', numios, length(current_types));
      |     end
      | end
      | problem = 0;
      | for ctr = 1 : numios,
      |     t = current_types(ctr);
      |     if (t < 0) || (t > 2),
      |         problem = t;
      |         ctr = numios + 1;
      |     end
      | end
      | if problem ~= 0,
      |     error('Type cannot be %i, must be 0, 1 or 2.', problem);
      | end
      mask Callback bin_pts:
      | blk = gcb;
      | mode = get_param(blk, 'mode');
      | current_bins = eval(get_param(blk, 'bin_pts'));
      | if (strcmp(mode, 'one value') || strcmp(mode, 'fields of equal size')) && (length(current_bins) > 1),
      |     error('Only one binary pt may be specified for this mode.');
      | elseif strcmp(mode, 'fields of arbitrary size')
      |     current_names = textscan(strtrim(strrep(strrep(get_param(blk, 'names'), ']', ''), '[', '')), '%s');
      |     current_names = current_names{1};
      |     numios = length(current_names);
      |     if length(current_bins) ~= numios,
      |         error('%d field names specified, but %d binary pts?', numios, length(current_bins));
      |     end
      | end
  wires:
  Subsystem5/1(rx_cnt) -> Delay66/1(d)
  [cnt_rst] -> Subsystem5/1(rst)
  miss_cnt0/2(missing_cnt) -> Convert1/1
  [cnt_rst] -> miss_cnt0/1(rst)
  Subsystem5/2(err_cnt) -> Delay67/1(d)
  miss_cnt0/1(spectr_cnt) -> Convert/1
  Delay61/1(q) -> pkt_reord_cnt0/1(out_reg)
  Delay62/1(q) -> pkt_reord_err0/1(out_reg)
  Delay66/1(q) -> rx_cnt0/1(out_reg)
  Delay67/1(q) -> rx_err_cnt0/1(out_reg)
  pkt_reord_devel0/4(time_out) -> Slice38/1, Delay26/1(d)
  pkt_reord_devel0/1(sync_out) -> Delay20/1(d), [x_sync0], snap_reord0/1(in_sync), snap_reord0/11(trig), delay61/1
  master_reset_sim4/1 -> acc_len/1(sim_1)
  acc_len/1(in_reg) -> [acc_len]
  [xeng_tvg_sel] -> Terminator1/1
  Delay20/1(q) -> Terminator3/1
  Delay21/1(q) -> Terminator5/1
  Delay130/1(q) -> last_missing_ant0/1(out_reg)
  miss_cnt0/3(last_missed_ant) -> Convert2/1
  [gbe_rxvld0] -> Delay6/1(d)
  [gbe_rxdata0] -> Delay2/1(d)
  [gbe_rxeof0] -> Delay7/1(d)
  Delay2/1(q) -> spead_unpack0/1(pkt_data)
  Delay6/1(q) -> spead_unpack0/2(pkt_valid)
  Delay7/1(q) -> spead_unpack0/3(pkt_eof)
  Delay80/1(q) -> Subsystem5/2(we)
  Delay81/1(q) -> Subsystem5/3(eof)
  Delay82/1(q) -> Subsystem5/4(flag)
  [gbe_rst] -> delay8/1
  [gbe_txd0] -> delay9/1
  [gbe_txvld0] -> delay10/1
  [gbe_txip] -> delay11/1
  [gbe_txport] -> delay12/1
  [gbe_txeof0] -> delay13/1
  gbe0/1(led_up) -> [gbe_up0]
  gbe0/2(led_rx) -> Terminator7/1
  gbe0/3(led_tx) -> Terminator13/1
  gbe0/4(tx_afull) -> Terminator14/1
  gbe0/5(tx_overflow) -> [gbe_tx_over0]
  gbe0/12(rx_overrun) -> Terminator36/1
  gbe0/11(rx_bad_frame) -> [gbe_rx_bad0]
  gbe0/6(rx_data) -> [gbe_rxdata0]
  gbe0/7(rx_valid) -> [gbe_rxvld0]
  gbe0/8(rx_source_ip) -> Terminator15/1
  gbe0/9(rx_source_port) -> Terminator35/1
  gbe0/10(rx_end_of_frame) -> [gbe_rxeof0]
  pkt_reord_devel0/2(data_out) -> snap_reord0/2(in_data), Delay21/1(d)
  miss_cnt0/4(not_rcvd) -> [xeng_rx_err0]
  delay8/1 -> gbe0/1(rst)
  delay9/1 -> gbe0/2(tx_data)
  delay10/1 -> gbe0/3(tx_valid)
  delay11/1 -> gbe0/4(tx_dest_ip)
  delay12/1 -> gbe0/5(tx_dest_port)
  delay13/1 -> gbe0/6(tx_end_of_frame)
  Constant2/1 -> gbe0/7(rx_ack)
  Constant8/1 -> gbe0/8(rx_overrun_ack)
  Constant22/1 -> [beng_data_id]
  gbe_porttx/1(in_reg) -> Delay9/1(d)
  gbe_iptx/1(in_reg) -> Delay10/1(d)
  Delay9/1(q) -> [gbe_txport]
  Delay10/1(q) -> [gbe_txip]
  Constant24/1 -> [beng_time_id]
  spead_unpack0/1(pkt_start) -> Terminator28/1
  pre_process0/9(dest_err) -> [pre_rx_dest_err0]
  pre_process0/1(data_out) -> [pre_data_0], pkt_reord_devel0/1(din)
  pre_process0/2(valid) -> [pre_valid_0], pkt_reord_devel0/2(valid_in)
  pre_process0/3(eof_out) -> [pre_eof_0], pkt_reord_devel0/3(eof)
  pre_process0/4(timestamp) -> [pre_timestamp_0], pkt_reord_devel0/4(time)
  pre_process0/5(feng_id) -> [pre_feng_id_0], pkt_reord_devel0/5(ant)
  pre_process0/6(freq_out) -> [pre_freq_0], pkt_reord_devel0/6(freq)
  pre_process0/8(spead_err_out) -> [pre_spead_err0]
  pre_process0/7(adc_over) -> [pre_adc_err0]
  pre_process0/10(fft_err) -> [pre_fft_err0]
  pre_process0/11(feng_rx_err) -> [pre_feng_rx_err0]
  pre_process0/12(nd_en) -> [pre_ndiode_en0]
  pkt_reord_devel0/7(err) -> Terminator2/1
  pre_process0/13(chksum_err) -> [pre_feng_chk_err0]
  pre_process0/14(qdr_err) -> [pre_feng_qdr_err0]
  [id0] -> pre_process0/9(board_id)
  board_id/1(in_reg) -> Delay72/1(d)
  Delay72/1(q) -> Subsystem1/1(In1)
  Subsystem1/1(Out1) -> [id0]
  Subsystem1/2(Out2) -> [id1]
  Subsystem1/3(Out3) -> [id2]
  Subsystem1/4(Out4) -> [id3]
  [id0] -> pkt_reord_devel0/8(board_id)
  pkt_reord_devel0/3(valid_out) -> delay62/1, snap_reord0/3(in_valid), snap_reord0/10(we), Logical6/2, Delay22/1(d)
  pkt_reord_devel0/5(freq_out) -> Convert12/1
  Slice12/1 -> snap_reord0/7(in_feng_err)
  Slice16/1 -> snap_reord0/9(in_nd_on)
  Slice15/1 -> snap_reord0/8(in_adc_over)
  pkt_reord_devel0/6(flag_out) -> Slice11/1, Slice12/1, Slice15/1, Slice16/1
  Slice11/1 -> snap_reord0/6(in_xeng_err), Logical6/1, delay63/1
  Logical6/1 -> snap_reord0/12(stop)
  Constant6/1 -> vacc_time_lsw/1(sim_1)
  vacc_time_msw/2(in_msw) -> Concat12/1
  vacc_time_lsw/1(in_reg) -> Concat12/2
  vacc_time_msw/1(in_arm) -> [vacc_ld_arm]
  Concat12/1 -> [vacc_ld_time]
  [gbe_rst] -> delay21/1
  [gbe_txd1] -> delay22/1
  [gbe_txip] -> delay15/1
  [gbe_txport] -> delay19/1
  delay21/1 -> gbe1/1(rst)
  delay22/1 -> gbe1/2(tx_data)
  delay14/1 -> gbe1/3(tx_valid)
  delay15/1 -> gbe1/4(tx_dest_ip)
  delay19/1 -> gbe1/5(tx_dest_port)
  delay20/1 -> gbe1/6(tx_end_of_frame)
  Constant9/1 -> gbe1/7(rx_ack)
  Constant13/1 -> gbe1/8(rx_overrun_ack)
  gbe1/11(rx_bad_frame) -> [gbe_rx_bad1]
  gbe1/5(tx_overflow) -> [gbe_tx_over1]
  [gbe_txeof1] -> delay20/1
  [gbe_txvld1] -> delay14/1
  gbe1/1(led_up) -> [gbe_up1]
  [flags0] -> pkt_reord_devel0/7(flag)
  Slice38/1 -> snap_reord0/4(in_time)
  Convert12/1 -> snap_reord0/5(in_freq)
  Convert/1 -> Delay61/1(d)
  Convert1/1 -> Delay62/1(d)
  Convert2/1 -> Delay130/1(d)
  control/3(in_cnt_rst) -> edge_detect/1(in)
  control/1(in_vacc_rst) -> edge_detect2/1(in)
  control/2(in_clr_status) -> edge_detect3/1(in)
  control/4(in_gbe_rst) -> pipeline4/1(d)
  control/7(in_loopback_rst) -> edge_detect4/1(in)
  control/8(in_flasher_en) -> pipeline8/1(d)
  edge_detect/1(out) -> pipeline2/1(d)
  pipeline8/1(q) -> [flasher_en]
  pipeline7/1(q) -> [loopback_mux_rst]
  pipeline5/1(q) -> [gbe_txen]
  pipeline4/1(q) -> [gbe_rst]
  pipeline2/1(q) -> [cnt_rst]
  pipeline1/1(q) -> [clr_status]
  pipeline/1(q) -> [vacc_rst]
  tvg_select/1(in_xaui) -> pipeline9/1(d)
  tvg_select/3(in_xeng) -> pipeline12/1(d)
  tvg_select/4(in_vacc) -> pipeline11/1(d)
  pipeline9/1(q) -> [xaui_tvg_sel]
  pipeline10/1(q) -> [descr_tvg_sel]
  pipeline12/1(q) -> [xeng_tvg_sel]
  pipeline11/1(q) -> [vacc_tvg_sel]
  pipeline13/1(q) -> [gbe_debug_rst]
  control/6(in_gbe_debug_rst) -> edge_detect1/1(in)
  [gbe_debug_rst] -> gbe0/9(debug_rst)
  [gbe_debug_rst] -> gbe1/9(debug_rst)
  gbe1/2(led_rx) -> Terminator38/1
  gbe1/3(led_tx) -> Terminator50/1
  gbe1/4(tx_afull) -> Terminator51/1
  gbe1/8(rx_source_ip) -> Terminator52/1
  gbe1/9(rx_source_port) -> Terminator53/1
  gbe1/12(rx_overrun) -> Terminator54/1
  gbe1/6(rx_data) -> [gbe_rxdata1]
  gbe1/7(rx_valid) -> [gbe_rxvld1]
  gbe1/10(rx_end_of_frame) -> [gbe_rxeof1]
  tvg_select/2(in_descramble) -> pipeline10/1(d)
  control/5(in_gbe_txen) -> pipeline5/1(d)
  Constant1/1 -> [flags2], [flags3], [flags1], [flags0]
  Constant3/1 -> [gbe_txvld1], [gbe_txvld0]
  Constant4/1 -> [gbe_txd1], [gbe_txd0]
  Constant5/1 -> [gbe_txeof1], [gbe_txeof0]
  edge_detect1/1(out) -> pipeline13/1(d)
  [spead_valid0] -> Delay80/1(d)
  [spead_eof0] -> Delay81/1(d)
  [spead_error0] -> Delay82/1(d)
  spead_unpack0/2(data64) -> [spead_data0]
  spead_unpack0/3(valid64) -> [spead_valid0]
  spead_unpack0/4(eof64) -> [spead_eof0]
  spead_unpack0/5(error) -> [spead_error0]
  spead_unpack0/6(hdr_heap_id) -> [spead_heapid0]
  spead_unpack0/7(hdr_heap_size) -> [spead_heapsize0]
  spead_unpack0/8(hdr_heap_offset) -> [spead_heapoffset0]
  spead_unpack0/9(hdr_pkt_len) -> [spead_pktlen0]
  spead_unpack0/10(hdr5_0x1600) -> [spead_hdr1_0]
  spead_unpack0/11(hdr6_0x4101) -> [spead_hdr2_0]
  spead_unpack0/12(hdr7_0x4102) -> [spead_hdr3_0]
  spead_unpack0/13(hdr8_0x4103) -> [spead_hdr4_0]
  [spead_data0] -> pre_process0/1(data_in)
  [spead_valid0] -> pre_process0/2(valid_in)
  [spead_eof0] -> pre_process0/3(eof_in)
  [spead_error0] -> pre_process0/4(spead_err)
  [spead_hdr1_0] -> pre_process0/5(hdr1)
  [spead_hdr2_0] -> pre_process0/6(hdr2)
  [spead_hdr3_0] -> pre_process0/7(hdr3)
  [spead_hdr4_0] -> pre_process0/8(hdr4)
  Slice1/1 -> snap_unpack0/4(in_time)
  Slice2/1 -> snap_unpack0/5(in_feng_id)
  Slice3/1 -> snap_unpack0/6(in_freq)
  Logical2/1 -> snap_unpack0/17(stop)
  [pre_valid_0] -> snap_unpack0/15(we), snap_unpack0/2(in_valid)
  [pre_eof_0] -> snap_unpack0/16(trig), snap_unpack0/3(in_eof)
  [pre_timestamp_0] -> Slice1/1
  [pre_feng_id_0] -> Slice2/1
  [pre_freq_0] -> Slice3/1
  [pre_data_0] -> snap_unpack0/1(in_data)
  [pre_spead_err0] -> Logical2/1
  [pre_rx_dest_err0] -> Logical2/2
  [pre_feng_rx_err0] -> Logical2/3
  [pre_feng_chk_err0] -> Logical2/4
  [pre_feng_rx_err0] -> snap_unpack0/11(in_feng_rx_err)
  [pre_adc_err0] -> snap_unpack0/7(in_adc_over)
  [pre_spead_err0] -> snap_unpack0/8(in_spead_err)
  [pre_rx_dest_err0] -> snap_unpack0/9(in_dest_err)
  [pre_fft_err0] -> snap_unpack0/10(in_fft_err)
  [pre_ndiode_en0] -> snap_unpack0/12(in_nd_en)
  [pre_feng_chk_err0] -> snap_unpack0/13(in_chksum_err)
  [pre_feng_qdr_err0] -> snap_unpack0/14(in_feng_qdr_err)
  Delay22/1(q) -> Terminator4/1
  Delay26/1(q) -> Terminator6/1
  miss_cnt1/2(missing_cnt) -> Convert4/1
  [cnt_rst] -> miss_cnt1/1(rst)
  miss_cnt1/1(spectr_cnt) -> Convert3/1
  Delay11/1(q) -> pkt_reord_cnt1/1(out_reg)
  Delay12/1(q) -> pkt_reord_err1/1(out_reg)
  pkt_reord_devel1/4(time_out) -> Delay8/1(d)
  pkt_reord_devel1/1(sync_out) -> delay64/1, [x_sync1], Delay3/1(d)
  [xeng_tvg_sel] -> Terminator8/1
  Delay3/1(q) -> Terminator10/1
  Delay4/1(q) -> Terminator12/1
  Delay1/1(q) -> last_missing_ant1/1(out_reg)
  miss_cnt1/3(last_missed_ant) -> Convert6/1
  pkt_reord_devel1/2(data_out) -> Delay4/1(d)
  miss_cnt1/4(not_rcvd) -> [xeng_rx_err1]
  pre_process1/9(dest_err) -> [pre_rx_dest_err1]
  pre_process1/1(data_out) -> pkt_reord_devel1/1(din), [pre_data_1]
  pre_process1/2(valid) -> pkt_reord_devel1/2(valid_in), [pre_valid_1]
  pre_process1/3(eof_out) -> pkt_reord_devel1/3(eof), [pre_eof_1]
  pre_process1/4(timestamp) -> pkt_reord_devel1/4(time), [pre_timestamp_1]
  pre_process1/5(feng_id) -> pkt_reord_devel1/5(ant), [pre_feng_id_1]
  pre_process1/6(freq_out) -> pkt_reord_devel1/6(freq), [pre_freq_1]
  pre_process1/8(spead_err_out) -> [pre_spead_err1]
  pre_process1/7(adc_over) -> [pre_adc_err1]
  pre_process1/10(fft_err) -> [pre_fft_err1]
  pre_process1/11(feng_rx_err) -> [pre_feng_rx_err1]
  pre_process1/12(nd_en) -> [pre_ndiode_en1]
  pkt_reord_devel1/7(err) -> Terminator9/1
  pre_process1/13(chksum_err) -> [pre_feng_chk_err1]
  pre_process1/14(qdr_err) -> [pre_feng_qdr_err1]
  [id1] -> pre_process1/9(board_id)
  [id1] -> pkt_reord_devel1/8(board_id)
  pkt_reord_devel1/3(valid_out) -> Delay5/1(d), delay65/1
  pkt_reord_devel1/6(flag_out) -> Slice4/1
  Slice4/1 -> delay66/1
  [flags1] -> pkt_reord_devel1/7(flag)
  Convert3/1 -> Delay11/1(d)
  Convert4/1 -> Delay12/1(d)
  Convert6/1 -> Delay1/1(d)
  [spead_data0] -> pre_process1/1(data_in)
  [spead_valid0] -> pre_process1/2(valid_in)
  [spead_eof0] -> pre_process1/3(eof_in)
  [spead_error0] -> pre_process1/4(spead_err)
  [spead_hdr1_0] -> pre_process1/5(hdr1)
  [spead_hdr2_0] -> pre_process1/6(hdr2)
  [spead_hdr3_0] -> pre_process1/7(hdr3)
  [spead_hdr4_0] -> pre_process1/8(hdr4)
  Delay5/1(q) -> Terminator11/1
  Delay8/1(q) -> Terminator16/1
  Subsystem3/1(rx_cnt) -> Delay32/1(d)
  [cnt_rst] -> Subsystem3/1(rst)
  miss_cnt2/2(missing_cnt) -> Convert8/1
  [cnt_rst] -> miss_cnt2/1(rst)
  Subsystem3/2(err_cnt) -> Delay33/1(d)
  miss_cnt2/1(spectr_cnt) -> Convert7/1
  Delay30/1(q) -> pkt_reord_cnt2/1(out_reg)
  Delay31/1(q) -> pkt_reord_err2/1(out_reg)
  Delay32/1(q) -> rx_cnt1/1(out_reg)
  Delay33/1(q) -> rx_err_cnt1/1(out_reg)
  pkt_reord_devel2/4(time_out) -> Delay24/1(d)
  pkt_reord_devel2/1(sync_out) -> delay67/1, [x_sync2], Delay18/1(d)
  [xeng_tvg_sel] -> Terminator17/1
  Delay18/1(q) -> Terminator24/1
  Delay19/1(q) -> Terminator26/1
  Delay16/1(q) -> last_missing_ant2/1(out_reg)
  miss_cnt2/3(last_missed_ant) -> Convert10/1
  [gbe_rxvld1] -> Delay29/1(d)
  [gbe_rxdata1] -> Delay17/1(d)
  [gbe_rxeof1] -> Delay34/1(d)
  Delay17/1(q) -> spead_unpack1/1(pkt_data)
  Delay29/1(q) -> spead_unpack1/2(pkt_valid)
  Delay34/1(q) -> spead_unpack1/3(pkt_eof)
  Delay36/1(q) -> Subsystem3/2(we)
  Delay37/1(q) -> Subsystem3/3(eof)
  Delay38/1(q) -> Subsystem3/4(flag)
  pkt_reord_devel2/2(data_out) -> Delay19/1(d)
  miss_cnt2/4(not_rcvd) -> [xeng_rx_err2]
  spead_unpack1/1(pkt_start) -> Terminator23/1
  pre_process2/9(dest_err) -> [pre_rx_dest_err2]
  pre_process2/1(data_out) -> pkt_reord_devel2/1(din), [pre_data_2]
  pre_process2/2(valid) -> pkt_reord_devel2/2(valid_in), [pre_valid_2]
  pre_process2/3(eof_out) -> pkt_reord_devel2/3(eof), [pre_eof_2]
  pre_process2/4(timestamp) -> pkt_reord_devel2/4(time), [pre_timestamp_2]
  pre_process2/5(feng_id) -> pkt_reord_devel2/5(ant), [pre_feng_id_2]
  pre_process2/6(freq_out) -> pkt_reord_devel2/6(freq), [pre_freq_2]
  pre_process2/8(spead_err_out) -> [pre_spead_err2]
  pre_process2/7(adc_over) -> [pre_adc_err2]
  pre_process2/10(fft_err) -> [pre_fft_err2]
  pre_process2/11(feng_rx_err) -> [pre_feng_rx_err2]
  pre_process2/12(nd_en) -> [pre_ndiode_en2]
  pkt_reord_devel2/7(err) -> Terminator22/1
  pre_process2/13(chksum_err) -> [pre_feng_chk_err2]
  pre_process2/14(qdr_err) -> [pre_feng_qdr_err2]
  [id2] -> pre_process2/9(board_id)
  [id2] -> pkt_reord_devel2/8(board_id)
  pkt_reord_devel2/3(valid_out) -> delay68/1, Delay23/1(d)
  pkt_reord_devel2/6(flag_out) -> Slice9/1
  Slice9/1 -> delay69/1
  [flags2] -> pkt_reord_devel2/7(flag)
  Convert7/1 -> Delay30/1(d)
  Convert8/1 -> Delay31/1(d)
  Convert10/1 -> Delay16/1(d)
  [spead_valid1] -> Delay36/1(d)
  [spead_eof1] -> Delay37/1(d)
  [spead_error1] -> Delay38/1(d)
  spead_unpack1/2(data64) -> [spead_data1]
  spead_unpack1/3(valid64) -> [spead_valid1]
  spead_unpack1/4(eof64) -> [spead_eof1]
  spead_unpack1/5(error) -> [spead_error1]
  spead_unpack1/6(hdr_heap_id) -> [spead_heapid1]
  spead_unpack1/7(hdr_heap_size) -> [spead_heapsize1]
  spead_unpack1/8(hdr_heap_offset) -> [spead_heapoffset1]
  spead_unpack1/9(hdr_pkt_len) -> [spead_pktlen1]
  spead_unpack1/10(hdr5_0x1600) -> [spead_hdr1_1]
  spead_unpack1/11(hdr6_0x4101) -> [spead_hdr2_1]
  spead_unpack1/12(hdr7_0x4102) -> [spead_hdr3_1]
  spead_unpack1/13(hdr8_0x4103) -> [spead_hdr4_1]
  [spead_data1] -> pre_process2/1(data_in)
  [spead_valid1] -> pre_process2/2(valid_in)
  [spead_eof1] -> pre_process2/3(eof_in)
  [spead_error1] -> pre_process2/4(spead_err)
  [spead_hdr1_1] -> pre_process2/5(hdr1)
  [spead_hdr2_1] -> pre_process2/6(hdr2)
  [spead_hdr3_1] -> pre_process2/7(hdr3)
  [spead_hdr4_1] -> pre_process2/8(hdr4)
  Delay23/1(q) -> Terminator25/1
  Delay24/1(q) -> Terminator27/1
  miss_cnt3/2(missing_cnt) -> Convert13/1
  [cnt_rst] -> miss_cnt3/1(rst)
  miss_cnt3/1(spectr_cnt) -> Convert11/1
  Delay14/1(q) -> pkt_reord_cnt3/1(out_reg)
  Delay15/1(q) -> pkt_reord_err3/1(out_reg)
  pkt_reord_devel3/4(time_out) -> Delay35/1(d)
  pkt_reord_devel3/1(sync_out) -> Delay25/1(d), [x_sync3], delay70/1
  [xeng_tvg_sel] -> Terminator29/1
  Delay25/1(q) -> Terminator18/1
  Delay27/1(q) -> Terminator20/1
  Delay13/1(q) -> last_missing_ant3/1(out_reg)
  miss_cnt3/3(last_missed_ant) -> Convert15/1
  pkt_reord_devel3/2(data_out) -> Delay27/1(d)
  miss_cnt3/4(not_rcvd) -> [xeng_rx_err3]
  pre_process3/9(dest_err) -> [pre_rx_dest_err3]
  pre_process3/1(data_out) -> [pre_data_3], pkt_reord_devel3/1(din)
  pre_process3/2(valid) -> [pre_valid_3], pkt_reord_devel3/2(valid_in)
  pre_process3/3(eof_out) -> [pre_eof_3], pkt_reord_devel3/3(eof)
  pre_process3/4(timestamp) -> [pre_timestamp_3], pkt_reord_devel3/4(time)
  pre_process3/5(feng_id) -> [pre_feng_id_3], pkt_reord_devel3/5(ant)
  pre_process3/6(freq_out) -> [pre_freq_3], pkt_reord_devel3/6(freq)
  pre_process3/8(spead_err_out) -> [pre_spead_err3]
  pre_process3/7(adc_over) -> [pre_adc_err3]
  pre_process3/10(fft_err) -> [pre_fft_err3]
  pre_process3/11(feng_rx_err) -> [pre_feng_rx_err3]
  pre_process3/12(nd_en) -> [pre_ndiode_en3]
  pkt_reord_devel3/7(err) -> Terminator30/1
  pre_process3/13(chksum_err) -> [pre_feng_chk_err3]
  pre_process3/14(qdr_err) -> [pre_feng_qdr_err3]
  [id3] -> pre_process3/9(board_id)
  [id3] -> pkt_reord_devel3/8(board_id)
  pkt_reord_devel3/3(valid_out) -> delay71/1, Delay28/1(d)
  pkt_reord_devel3/6(flag_out) -> Slice18/1
  Slice18/1 -> delay72/1
  [flags3] -> pkt_reord_devel3/7(flag)
  Convert11/1 -> Delay14/1(d)
  Convert13/1 -> Delay15/1(d)
  Convert15/1 -> Delay13/1(d)
  [spead_data1] -> pre_process3/1(data_in)
  [spead_valid1] -> pre_process3/2(valid_in)
  [spead_eof1] -> pre_process3/3(eof_in)
  [spead_error1] -> pre_process3/4(spead_err)
  [spead_hdr1_1] -> pre_process3/5(hdr1)
  [spead_hdr2_1] -> pre_process3/6(hdr2)
  [spead_hdr3_1] -> pre_process3/7(hdr3)
  [spead_hdr4_1] -> pre_process3/8(hdr4)
  Delay28/1(q) -> Terminator19/1
  Delay35/1(q) -> Terminator21/1
  edge_detect2/1(out) -> pipeline/1(d)
  edge_detect3/1(out) -> pipeline1/1(d)
  edge_detect4/1(out) -> pipeline7/1(d)
  Slice5/1 -> snap_unpack1/4(in_time)
  Slice6/1 -> snap_unpack1/5(in_feng_id)
  Slice7/1 -> snap_unpack1/6(in_freq)
  Logical1/1 -> snap_unpack1/17(stop)
  [pre_valid_1] -> snap_unpack1/15(we), snap_unpack1/2(in_valid)
  [pre_eof_1] -> snap_unpack1/16(trig), snap_unpack1/3(in_eof)
  [pre_timestamp_1] -> Slice5/1
  [pre_feng_id_1] -> Slice6/1
  [pre_freq_1] -> Slice7/1
  [pre_data_1] -> snap_unpack1/1(in_data)
  [pre_spead_err1] -> Logical1/1
  [pre_rx_dest_err1] -> Logical1/2
  [pre_feng_rx_err1] -> Logical1/3
  [pre_feng_chk_err1] -> Logical1/4
  [pre_feng_rx_err1] -> snap_unpack1/11(in_feng_rx_err)
  [pre_adc_err1] -> snap_unpack1/7(in_adc_over)
  [pre_spead_err1] -> snap_unpack1/8(in_spead_err)
  [pre_rx_dest_err1] -> snap_unpack1/9(in_dest_err)
  [pre_fft_err1] -> snap_unpack1/10(in_fft_err)
  [pre_ndiode_en1] -> snap_unpack1/12(in_nd_en)
  [pre_feng_chk_err1] -> snap_unpack1/13(in_chksum_err)
  [pre_feng_qdr_err1] -> snap_unpack1/14(in_feng_qdr_err)
  Slice8/1 -> snap_unpack2/4(in_time)
  Slice10/1 -> snap_unpack2/5(in_feng_id)
  Slice13/1 -> snap_unpack2/6(in_freq)
  Logical3/1 -> snap_unpack2/17(stop)
  [pre_valid_2] -> snap_unpack2/15(we), snap_unpack2/2(in_valid)
  [pre_eof_2] -> snap_unpack2/16(trig), snap_unpack2/3(in_eof)
  [pre_timestamp_2] -> Slice8/1
  [pre_feng_id_2] -> Slice10/1
  [pre_freq_2] -> Slice13/1
  [pre_data_2] -> snap_unpack2/1(in_data)
  [pre_spead_err2] -> Logical3/1
  [pre_rx_dest_err2] -> Logical3/2
  [pre_feng_rx_err2] -> Logical3/3
  [pre_feng_chk_err2] -> Logical3/4
  [pre_feng_rx_err2] -> snap_unpack2/11(in_feng_rx_err)
  [pre_adc_err2] -> snap_unpack2/7(in_adc_over)
  [pre_spead_err2] -> snap_unpack2/8(in_spead_err)
  [pre_rx_dest_err2] -> snap_unpack2/9(in_dest_err)
  [pre_fft_err2] -> snap_unpack2/10(in_fft_err)
  [pre_ndiode_en2] -> snap_unpack2/12(in_nd_en)
  [pre_feng_chk_err2] -> snap_unpack2/13(in_chksum_err)
  [pre_feng_qdr_err2] -> snap_unpack2/14(in_feng_qdr_err)
  Slice14/1 -> snap_unpack3/4(in_time)
  Slice17/1 -> snap_unpack3/5(in_feng_id)
  Slice19/1 -> snap_unpack3/6(in_freq)
  Logical4/1 -> snap_unpack3/17(stop)
  [pre_valid_3] -> snap_unpack3/15(we), snap_unpack3/2(in_valid)
  [pre_eof_3] -> snap_unpack3/16(trig), snap_unpack3/3(in_eof)
  [pre_timestamp_3] -> Slice14/1
  [pre_feng_id_3] -> Slice17/1
  [pre_freq_3] -> Slice19/1
  [pre_data_3] -> snap_unpack3/1(in_data)
  [pre_spead_err3] -> Logical4/1
  [pre_rx_dest_err3] -> Logical4/2
  [pre_feng_rx_err3] -> Logical4/3
  [pre_feng_chk_err3] -> Logical4/4
  [pre_feng_rx_err3] -> snap_unpack3/11(in_feng_rx_err)
  [pre_adc_err3] -> snap_unpack3/7(in_adc_over)
  [pre_spead_err3] -> snap_unpack3/8(in_spead_err)
  [pre_rx_dest_err3] -> snap_unpack3/9(in_dest_err)
  [pre_fft_err3] -> snap_unpack3/10(in_fft_err)
  [pre_ndiode_en3] -> snap_unpack3/12(in_nd_en)
  [pre_feng_chk_err3] -> snap_unpack3/13(in_chksum_err)
  [pre_feng_qdr_err3] -> snap_unpack3/14(in_feng_qdr_err)
  [cnt_rst] -> delay1/1
  [pre_freq_0] -> Slice/1
  Constant/1 -> Relational/2
  [pre_feng_id_0] -> Slice20/1
  Relational/1 -> Logical5/2
  Logical5/1 -> delay7/1
  [cnt_rst] -> delay2/1
  Constant7/1 -> Relational1/2
  Relational1/1 -> Logical7/2
  Logical7/1 -> delay16/1
  [cnt_rst] -> delay3/1
  Constant10/1 -> Relational2/2
  Relational2/1 -> Logical8/2
  Logical8/1 -> delay18/1
  [cnt_rst] -> delay4/1
  Constant11/1 -> Relational3/2
  Relational3/1 -> Logical9/2
  [pre_valid_0] -> Logical9/1, Logical8/1, Logical7/1, Logical5/1
  Logical9/1 -> delay24/1
  Convert5/1 -> Delay39/1(d)
  highwater16/1(highmark) -> Convert5/1
  Delay39/1(q) -> highmark0_01/1(out_high0)
  Convert9/1 -> Delay40/1(d)
  Delay40/1(q) -> highmark0_01/2(out_high1)
  highwater1/1(highmark) -> Convert9/1
  Convert14/1 -> Delay41/1(d)
  Convert16/1 -> Delay42/1(d)
  highwater2/1(highmark) -> Convert14/1
  Delay41/1(q) -> highmark0_23/1(out_high2)
  Delay42/1(q) -> highmark0_23/2(out_high3)
  highwater3/1(highmark) -> Convert16/1
  delay1/1 -> highwater16/1(reset)
  delay2/1 -> highwater1/1(reset)
  delay3/1 -> highwater2/1(reset)
  delay4/1 -> highwater3/1(reset)
  delay5/1 -> highwater16/3(data)
  delay7/1 -> highwater16/2(valid)
  delay16/1 -> highwater1/2(valid)
  delay17/1 -> highwater1/3(data)
  delay18/1 -> highwater2/2(valid)
  delay23/1 -> highwater2/3(data)
  delay24/1 -> highwater3/2(valid)
  delay25/1 -> highwater3/3(data)
  Slice/1 -> delay25/1, delay23/1, delay17/1, delay5/1
  Slice20/1 -> Relational/1, Relational3/1, Relational2/1, Relational1/1
  [id0] -> highwater3/4(xid), highwater2/4(xid), highwater1/4(xid), highwater16/4(xid)
  [cnt_rst] -> delay6/1
  [pre_freq_1] -> Slice21/1
  Constant12/1 -> Relational4/2
  [pre_feng_id_1] -> Slice22/1
  Relational4/1 -> Logical10/2
  Logical10/1 -> delay36/1
  [cnt_rst] -> delay29/1
  Constant16/1 -> Relational5/2
  Relational5/1 -> Logical11/2
  Logical11/1 -> delay26/1
  [cnt_rst] -> delay33/1
  Constant14/1 -> Relational6/2
  Relational6/1 -> Logical12/2
  Logical12/1 -> delay28/1
  [cnt_rst] -> delay34/1
  Constant15/1 -> Relational7/2
  Relational7/1 -> Logical13/2
  [pre_valid_1] -> Logical10/1, Logical11/1, Logical12/1, Logical13/1
  Logical13/1 -> delay31/1
  Convert19/1 -> Delay43/1(d)
  highwater5/1(highmark) -> Convert19/1
  Delay43/1(q) -> highmark1_01/1(out_high0)
  Convert20/1 -> Delay44/1(d)
  Delay44/1(q) -> highmark1_01/2(out_high1)
  highwater4/1(highmark) -> Convert20/1
  Convert17/1 -> Delay45/1(d)
  Convert18/1 -> Delay46/1(d)
  highwater6/1(highmark) -> Convert17/1
  Delay45/1(q) -> highmark1_23/1(out_high2)
  Delay46/1(q) -> highmark1_23/2(out_high3)
  highwater7/1(highmark) -> Convert18/1
  delay6/1 -> highwater5/1(reset)
  delay29/1 -> highwater4/1(reset)
  delay33/1 -> highwater6/1(reset)
  delay34/1 -> highwater7/1(reset)
  delay35/1 -> highwater5/3(data)
  delay36/1 -> highwater5/2(valid)
  delay26/1 -> highwater4/2(valid)
  delay27/1 -> highwater4/3(data)
  delay28/1 -> highwater6/2(valid)
  delay30/1 -> highwater6/3(data)
  delay31/1 -> highwater7/2(valid)
  delay32/1 -> highwater7/3(data)
  Slice21/1 -> delay35/1, delay27/1, delay30/1, delay32/1
  Slice22/1 -> Relational5/1, Relational6/1, Relational7/1, Relational4/1
  [id1] -> highwater7/4(xid), highwater6/4(xid), highwater4/4(xid), highwater5/4(xid)
  [cnt_rst] -> delay48/1
  [pre_freq_2] -> Slice23/1
  Constant17/1 -> Relational8/2
  [pre_feng_id_2] -> Slice24/1
  Relational8/1 -> Logical14/2
  Logical14/1 -> delay47/1
  [cnt_rst] -> delay40/1
  Constant20/1 -> Relational9/2
  Relational9/1 -> Logical15/2
  Logical15/1 -> delay37/1
  [cnt_rst] -> delay44/1
  Constant18/1 -> Relational10/2
  Relational10/1 -> Logical16/2
  Logical16/1 -> delay39/1
  [cnt_rst] -> delay45/1
  Constant19/1 -> Relational11/2
  Relational11/1 -> Logical17/2
  [pre_valid_2] -> Logical17/1, Logical16/1, Logical15/1, Logical14/1
  Logical17/1 -> delay42/1
  Convert23/1 -> Delay47/1(d)
  highwater9/1(highmark) -> Convert23/1
  Delay47/1(q) -> highmark2_01/1(out_high0)
  Convert24/1 -> Delay48/1(d)
  Delay48/1(q) -> highmark2_01/2(out_high1)
  highwater8/1(highmark) -> Convert24/1
  Convert21/1 -> Delay49/1(d)
  Convert22/1 -> Delay50/1(d)
  highwater10/1(highmark) -> Convert21/1
  Delay49/1(q) -> highmark2_23/1(out_high2)
  Delay50/1(q) -> highmark2_23/2(out_high3)
  highwater11/1(highmark) -> Convert22/1
  delay48/1 -> highwater9/1(reset)
  delay40/1 -> highwater8/1(reset)
  delay44/1 -> highwater10/1(reset)
  delay45/1 -> highwater11/1(reset)
  delay46/1 -> highwater9/3(data)
  delay47/1 -> highwater9/2(valid)
  delay37/1 -> highwater8/2(valid)
  delay38/1 -> highwater8/3(data)
  delay39/1 -> highwater10/2(valid)
  delay41/1 -> highwater10/3(data)
  delay42/1 -> highwater11/2(valid)
  delay43/1 -> highwater11/3(data)
  Slice23/1 -> delay43/1, delay41/1, delay38/1, delay46/1
  Slice24/1 -> Relational8/1, Relational11/1, Relational10/1, Relational9/1
  [id2] -> highwater11/4(xid), highwater10/4(xid), highwater8/4(xid), highwater9/4(xid)
  [cnt_rst] -> delay60/1
  [pre_freq_3] -> Slice25/1
  Constant21/1 -> Relational14/2
  [pre_feng_id_3] -> Slice26/1
  Relational14/1 -> Logical18/2
  Logical18/1 -> delay59/1
  [cnt_rst] -> delay52/1
  Constant26/1 -> Relational15/2
  Relational15/1 -> Logical19/2
  Logical19/1 -> delay49/1
  [cnt_rst] -> delay56/1
  Constant23/1 -> Relational12/2
  Relational12/1 -> Logical20/2
  Logical20/1 -> delay51/1
  [cnt_rst] -> delay57/1
  Constant25/1 -> Relational13/2
  Relational13/1 -> Logical21/2
  [pre_valid_3] -> Logical18/1, Logical19/1, Logical20/1, Logical21/1
  Logical21/1 -> delay54/1
  Convert27/1 -> Delay51/1(d)
  highwater15/1(highmark) -> Convert27/1
  Delay51/1(q) -> highmark3_01/1(out_high0)
  Convert28/1 -> Delay52/1(d)
  Delay52/1(q) -> highmark3_01/2(out_high1)
  highwater14/1(highmark) -> Convert28/1
  Convert25/1 -> Delay53/1(d)
  Convert26/1 -> Delay54/1(d)
  highwater12/1(highmark) -> Convert25/1
  Delay53/1(q) -> highmark3_23/1(out_high2)
  Delay54/1(q) -> highmark3_23/2(out_high3)
  highwater13/1(highmark) -> Convert26/1
  delay60/1 -> highwater15/1(reset)
  delay52/1 -> highwater14/1(reset)
  delay56/1 -> highwater12/1(reset)
  delay57/1 -> highwater13/1(reset)
  delay58/1 -> highwater15/3(data)
  delay59/1 -> highwater15/2(valid)
  delay49/1 -> highwater14/2(valid)
  delay50/1 -> highwater14/3(data)
  delay51/1 -> highwater12/2(valid)
  delay53/1 -> highwater12/3(data)
  delay54/1 -> highwater13/2(valid)
  delay55/1 -> highwater13/3(data)
  Slice25/1 -> delay58/1, delay50/1, delay53/1, delay55/1
  Slice26/1 -> Relational15/1, Relational12/1, Relational13/1, Relational14/1
  [id3] -> highwater13/4(xid), highwater12/4(xid), highwater14/4(xid), highwater15/4(xid)
  delay61/1 -> miss_cnt0/2(sync)
  delay62/1 -> miss_cnt0/3(valid)
  delay63/1 -> miss_cnt0/4(not rcvd)
  delay64/1 -> miss_cnt1/2(sync)
  delay65/1 -> miss_cnt1/3(valid)
  delay66/1 -> miss_cnt1/4(not rcvd)
  delay68/1 -> miss_cnt2/3(valid)
  delay69/1 -> miss_cnt2/4(not rcvd)
  delay67/1 -> miss_cnt2/2(sync)
  delay70/1 -> miss_cnt3/2(sync)
  delay72/1 -> miss_cnt3/4(not rcvd)
  delay71/1 -> miss_cnt3/3(valid)
